simulink model "model_compatible"  (Simulink 7.5)
(part 3 of 3)

  金剛線_(Kongō_sen)_CN_109834508_275000_CN_291678103_275000 : powerlib/Elements/Distributed Parameters Line  Phases=3  Frequency=50  Resistance=[0.01273 0.3864]  Inductance="[0.9337e-3  4.1264e-3]"  Capacitance=[12.74e-9 7.751e-9]  Length=50.4928  x1=[8.73114913702011e-11 380000 380000;314.159265358979 314.159265358979 314.159265358979;-0.177670123217348 0.415246442777429 -1.15554988401747]  x2=[1.26090477118469e-09 381852.398472139 381852.398472139;314.159265358979 314.159265358979 314.159265358979;-1.41941675517191 0.415007521738739 -1.15578880505616]  x3=[1.07663708898761e-11 1405.24743813465 1405.24743813466;314.159265358979 314.159265358979 314.159265358979;-2.70558821102223 0.316110507002444 -1.25468581979246]  x4=[8.62234243168895e-12 1405.96374414071 1405.9637441407;314.159265358979 314.159265358979 314.159265358979;0.245769282942371 0.405640215255436 -1.16515611153945]  x5=0.000565541566995742  V1=ones(3,3)  V2=ones(3,3)  I1=ones(3,3)  I2=ones(3,3)  nHarmo=1  Measurements=None
  関門連系線_CN_204258596_500000_CN_187988970_500000 : powerlib/Elements/Distributed Parameters Line  Phases=3  Frequency=50  Resistance=[0.01273 0.3864]  Inductance="[0.9337e-3  4.1264e-3]"  Capacitance=[12.74e-9 7.751e-9]  Length=77.4957  x1=[8.73114913702011e-11 380000 380000;314.159265358979 314.159265358979 314.159265358979;-0.177670123217348 0.415246442777429 -1.15554988401747]  x2=[1.26090477118469e-09 381852.398472139 381852.398472139;314.159265358979 314.159265358979 314.159265358979;-1.41941675517191 0.415007521738739 -1.15578880505616]  x3=[1.07663708898761e-11 1405.24743813465 1405.24743813466;314.159265358979 314.159265358979 314.159265358979;-2.70558821102223 0.316110507002444 -1.25468581979246]  x4=[8.62234243168895e-12 1405.96374414071 1405.9637441407;314.159265358979 314.159265358979 314.159265358979;0.245769282942371 0.405640215255436 -1.16515611153945]  x5=0.000565541566995742  V1=ones(3,3)  V2=ones(3,3)  I1=ones(3,3)  I2=ones(3,3)  nHarmo=1  Measurements=None
  阿南紀北直流幹線_CN_109850439_500000_CN_217885658_500000 : powerlib/Elements/Distributed Parameters Line  Phases=3  Frequency=50  Resistance=[0.01273 0.3864]  Inductance="[0.9337e-3  4.1264e-3]"  Capacitance=[12.74e-9 7.751e-9]  Length=61.602  x1=[8.73114913702011e-11 380000 380000;314.159265358979 314.159265358979 314.159265358979;-0.177670123217348 0.415246442777429 -1.15554988401747]  x2=[1.26090477118469e-09 381852.398472139 381852.398472139;314.159265358979 314.159265358979 314.159265358979;-1.41941675517191 0.415007521738739 -1.15578880505616]  x3=[1.07663708898761e-11 1405.24743813465 1405.24743813466;314.159265358979 314.159265358979 314.159265358979;-2.70558821102223 0.316110507002444 -1.25468581979246]  x4=[8.62234243168895e-12 1405.96374414071 1405.9637441407;314.159265358979 314.159265358979 314.159265358979;0.245769282942371 0.405640215255436 -1.16515611153945]  x5=0.000565541566995742  V1=ones(3,3)  V2=ones(3,3)  I1=ones(3,3)  I2=ones(3,3)  nHarmo=1  Measurements=None
  駿遠幹線_CN_116559939_500000_CN_210090094_500000 : powerlib/Elements/Distributed Parameters Line  Phases=3  Frequency=50  Resistance=[0.01273 0.3864]  Inductance="[0.9337e-3  4.1264e-3]"  Capacitance=[12.74e-9 7.751e-9]  Length=56.5258  x1=[8.73114913702011e-11 380000 380000;314.159265358979 314.159265358979 314.159265358979;-0.177670123217348 0.415246442777429 -1.15554988401747]  x2=[1.26090477118469e-09 381852.398472139 381852.398472139;314.159265358979 314.159265358979 314.159265358979;-1.41941675517191 0.415007521738739 -1.15578880505616]  x3=[1.07663708898761e-11 1405.24743813465 1405.24743813466;314.159265358979 314.159265358979 314.159265358979;-2.70558821102223 0.316110507002444 -1.25468581979246]  x4=[8.62234243168895e-12 1405.96374414071 1405.9637441407;314.159265358979 314.159265358979 314.159265358979;0.245769282942371 0.405640215255436 -1.16515611153945]  x5=0.000565541566995742  V1=ones(3,3)  V2=ones(3,3)  I1=ones(3,3)  I2=ones(3,3)  nHarmo=1  Measurements=None
  connections:
  _CN_201293312_500000_CN_216778426_500000/LConn1 -- T_201293312_500000;220000_/LConn1 -- _CN_201293312_500000_CN_187988970_500000/LConn1
  _CN_201293312_500000_CN_216778426_500000/LConn2 -- T_201293312_500000;220000_/LConn2 -- _CN_201293312_500000_CN_187988970_500000/LConn2
  _CN_201293312_500000_CN_216778426_500000/LConn3 -- T_201293312_500000;220000_/LConn3 -- _CN_201293312_500000_CN_187988970_500000/LConn3
  T_216778426_500000;220000_/LConn1 -- _CN_201293312_500000_CN_216778426_500000/RConn1
  T_216778426_500000;220000_/LConn2 -- _CN_201293312_500000_CN_216778426_500000/RConn2
  T_216778426_500000;220000_/LConn3 -- _CN_201293312_500000_CN_216778426_500000/RConn3
  _CN_201293312_500000_CN_187988970_500000/RConn1 -- T_187988970_500000;220000_/LConn1 -- 関門連系線_CN_204258596_500000_CN_187988970_500000/LConn1
  _CN_201293312_500000_CN_187988970_500000/RConn2 -- T_187988970_500000;220000_/LConn2 -- 関門連系線_CN_204258596_500000_CN_187988970_500000/LConn2
  _CN_201293312_500000_CN_187988970_500000/RConn3 -- T_187988970_500000;220000_/LConn3 -- 関門連系線_CN_204258596_500000_CN_187988970_500000/LConn3
  T_169121281__北豊田変電所_(Kita_Toyota_Hendensho)/LConn1 -- _CN_169121281_275000_CN_169121284_275000/LConn1
  T_169121281__北豊田変電所_(Kita_Toyota_Hendensho)/LConn2 -- _CN_169121281_275000_CN_169121284_275000/LConn2
  T_169121281__北豊田変電所_(Kita_Toyota_Hendensho)/LConn3 -- _CN_169121281_275000_CN_169121284_275000/LConn3
  _CN_169121281_275000_CN_169121284_275000/RConn1 -- T_169121284_275000_/LConn1 -- _CN_169121284_275000_CN_169121278_275000/LConn1
  _CN_169121281_275000_CN_169121284_275000/RConn2 -- T_169121284_275000_/LConn2 -- _CN_169121284_275000_CN_169121278_275000/LConn2
  _CN_169121281_275000_CN_169121284_275000/RConn3 -- T_169121284_275000_/LConn3 -- _CN_169121284_275000_CN_169121278_275000/LConn3
  T_104173570_500000_/LConn1 -- _CN_104173570_500000_CN_106309481_500000/LConn1
  T_104173570_500000_/LConn2 -- _CN_104173570_500000_CN_106309481_500000/LConn2
  T_104173570_500000_/LConn3 -- _CN_104173570_500000_CN_106309481_500000/LConn3
  _CN_104173570_500000_CN_106309481_500000/RConn1 -- T_106309481_500000_新福島変電所/LConn1 -- 福島東幹線2_CN_106309481_500000_CN_104391636_500000/LConn1 -- _CN_106309481_500000_CN103783431/LConn1
  _CN_104173570_500000_CN_106309481_500000/RConn2 -- T_106309481_500000_新福島変電所/LConn2 -- 福島東幹線2_CN_106309481_500000_CN_104391636_500000/LConn2 -- _CN_106309481_500000_CN103783431/LConn2
  _CN_104173570_500000_CN_106309481_500000/RConn3 -- T_106309481_500000_新福島変電所/LConn3 -- 福島東幹線2_CN_106309481_500000_CN_104391636_500000/LConn3 -- _CN_106309481_500000_CN103783431/LConn3
  T_116828675_275000_北相模変電所_(Kita_Sagami_Hendensho)/LConn1 -- 佐久間東幹線_CN_116828675_275000_CN134376414/LConn1
  T_116828675_275000_北相模変電所_(Kita_Sagami_Hendensho)/LConn2 -- 佐久間東幹線_CN_116828675_275000_CN134376414/LConn2
  T_116828675_275000_北相模変電所_(Kita_Sagami_Hendensho)/LConn3 -- 佐久間東幹線_CN_116828675_275000_CN134376414/LConn3
  G_134376414_佐久間発電所/RConn1 -- 佐久間東幹線_CN_116828675_275000_CN134376414/RConn1
  G_134376414_佐久間発電所/RConn2 -- 佐久間東幹線_CN_116828675_275000_CN134376414/RConn2
  G_134376414_佐久間発電所/RConn3 -- 佐久間東幹線_CN_116828675_275000_CN134376414/RConn3
  _CN_169121284_275000_CN_169121278_275000/RConn1 -- T_169121278_275000_電源名古屋/LConn1 -- _CN_170366038_275000_CN_169121278_275000/LConn1
  _CN_169121284_275000_CN_169121278_275000/RConn2 -- T_169121278_275000_電源名古屋/LConn2 -- _CN_170366038_275000_CN_169121278_275000/LConn2
  _CN_169121284_275000_CN_169121278_275000/RConn3 -- T_169121278_275000_電源名古屋/LConn3 -- _CN_170366038_275000_CN_169121278_275000/LConn3
  T_170503689__/LConn1 -- _CN_170503689_275000_CN_170436908_275000/LConn1
  T_170503689__/LConn2 -- _CN_170503689_275000_CN_170436908_275000/LConn2
  T_170503689__/LConn3 -- _CN_170503689_275000_CN_170436908_275000/LConn3
  T_170436908__/LConn1 -- _CN_170503689_275000_CN_170436908_275000/RConn1
  T_170436908__/LConn2 -- _CN_170503689_275000_CN_170436908_275000/RConn2
  T_170436908__/LConn3 -- _CN_170503689_275000_CN_170436908_275000/RConn3
  T_168857610__/LConn1 -- _CN_168857610_500000_CN_104530060_500000/LConn1
  T_168857610__/LConn2 -- _CN_168857610_500000_CN_104530060_500000/LConn2
  T_168857610__/LConn3 -- _CN_168857610_500000_CN_104530060_500000/LConn3
  _CN_168857610_500000_CN_104530060_500000/RConn1 -- T_104530060__新栃木変電所/LConn1 -- _CN_104530060_500000_CN_315434358_500000/LConn1 -- _CN_104530060_500000_CN_168839127_500000/LConn1
  _CN_168857610_500000_CN_104530060_500000/RConn2 -- T_104530060__新栃木変電所/LConn2 -- _CN_104530060_500000_CN_315434358_500000/LConn2 -- _CN_104530060_500000_CN_168839127_500000/LConn2
  _CN_168857610_500000_CN_104530060_500000/RConn3 -- T_104530060__新栃木変電所/LConn3 -- _CN_104530060_500000_CN_315434358_500000/LConn3 -- _CN_104530060_500000_CN_168839127_500000/LConn3
  _CN_193544791_500000_CN_170974371_500000/LConn1 -- T_193544791_500000_新西広島変電所_(Shin_Nishi_Hiroshima_Hendensho)/LConn1 -- _CN_193544791_500000_CN_242253500_500000/LConn1 -- _CN_193544791_500000_CN_317416612_500000/LConn1
  _CN_193544791_500000_CN_170974371_500000/LConn2 -- T_193544791_500000_新西広島変電所_(Shin_Nishi_Hiroshima_Hendensho)/LConn2 -- _CN_193544791_500000_CN_242253500_500000/LConn2 -- _CN_193544791_500000_CN_317416612_500000/LConn2
  _CN_193544791_500000_CN_170974371_500000/LConn3 -- T_193544791_500000_新西広島変電所_(Shin_Nishi_Hiroshima_Hendensho)/LConn3 -- _CN_193544791_500000_CN_242253500_500000/LConn3 -- _CN_193544791_500000_CN_317416612_500000/LConn3
  _CN_193544791_500000_CN_170974371_500000/RConn1 -- T_170974371_500000_新広島変電所_(Shin_Hiroshima_Hendensho)/LConn1 -- _CN_170974371_500000_CN_241828221_500000/LConn1
  _CN_193544791_500000_CN_170974371_500000/RConn2 -- T_170974371_500000_新広島変電所_(Shin_Hiroshima_Hendensho)/LConn2 -- _CN_170974371_500000_CN_241828221_500000/LConn2
  _CN_193544791_500000_CN_170974371_500000/RConn3 -- T_170974371_500000_新広島変電所_(Shin_Hiroshima_Hendensho)/LConn3 -- _CN_170974371_500000_CN_241828221_500000/LConn3
  _CN_193544791_500000_CN_242253500_500000/RConn1 -- T_242253500_500000_東山口変電所_(Higashi_Yamaguchi_Hendensho)/LConn1 -- _CN_242253500_500000_CN_204258596_500000/LConn1
  _CN_193544791_500000_CN_242253500_500000/RConn2 -- T_242253500_500000_東山口変電所_(Higashi_Yamaguchi_Hendensho)/LConn2 -- _CN_242253500_500000_CN_204258596_500000/LConn2
  _CN_193544791_500000_CN_242253500_500000/RConn3 -- T_242253500_500000_東山口変電所_(Higashi_Yamaguchi_Hendensho)/LConn3 -- _CN_242253500_500000_CN_204258596_500000/LConn3
  _CN_193544791_500000_CN_317416612_500000/RConn1 -- T_317416612_500000_西島根変電所/LConn1 -- _CN_317416612_500000_CN_204258596_500000/LConn1 -- _CN_317416612_500000_CN_242103481_500000/LConn1
  _CN_193544791_500000_CN_317416612_500000/RConn2 -- T_317416612_500000_西島根変電所/LConn2 -- _CN_317416612_500000_CN_204258596_500000/LConn2 -- _CN_317416612_500000_CN_242103481_500000/LConn2
  _CN_193544791_500000_CN_317416612_500000/RConn3 -- T_317416612_500000_西島根変電所/LConn3 -- _CN_317416612_500000_CN_204258596_500000/LConn3 -- _CN_317416612_500000_CN_242103481_500000/LConn3
  _CN_161727149_500000_CN_169031921_500000/LConn1 -- T_161727149_500000_新生駒変電所_(Shin_Ikoma_Hendensho)/LConn1 -- _CN_161727149_500000_CN_161870227_500000/LConn1 -- _CN_161727149_500000_CN_169359724_500000/LConn1
  _CN_161727149_500000_CN_169031921_500000/LConn2 -- T_161727149_500000_新生駒変電所_(Shin_Ikoma_Hendensho)/LConn2 -- _CN_161727149_500000_CN_161870227_500000/LConn2 -- _CN_161727149_500000_CN_169359724_500000/LConn2
  _CN_161727149_500000_CN_169031921_500000/LConn3 -- T_161727149_500000_新生駒変電所_(Shin_Ikoma_Hendensho)/LConn3 -- _CN_161727149_500000_CN_161870227_500000/LConn3 -- _CN_161727149_500000_CN_169359724_500000/LConn3
  _CN_161727149_500000_CN_169031921_500000/RConn1 -- T_169031921_500000_西京都変電所_(Nishi_Kyōto_Hendensho)/LConn1 -- _CN_320438391_500000_CN_169031921_500000/LConn1
  _CN_161727149_500000_CN_169031921_500000/RConn2 -- T_169031921_500000_西京都変電所_(Nishi_Kyōto_Hendensho)/LConn2 -- _CN_320438391_500000_CN_169031921_500000/LConn2
  _CN_161727149_500000_CN_169031921_500000/RConn3 -- T_169031921_500000_西京都変電所_(Nishi_Kyōto_Hendensho)/LConn3 -- _CN_320438391_500000_CN_169031921_500000/LConn3
  T_169359724_500000_信貴変電所_(Shingi_Hendensho)/LConn1 -- _CN_161727149_500000_CN_169359724_500000/RConn1
  T_169359724_500000_信貴変電所_(Shingi_Hendensho)/LConn2 -- _CN_161727149_500000_CN_169359724_500000/RConn2
  T_169359724_500000_信貴変電所_(Shingi_Hendensho)/LConn3 -- _CN_161727149_500000_CN_169359724_500000/RConn3
  _CN_161727149_500000_CN_161870227_500000/RConn1 -- T_161870227_500000_南京都変電所_(Minami_Kyōto_Hendensho)/LConn1 -- _CN_170589736_500000_CN_161870227_500000/LConn1 -- _CN_169031998_500000_CN_161870227_500000/LConn1
  _CN_161727149_500000_CN_161870227_500000/RConn2 -- T_161870227_500000_南京都変電所_(Minami_Kyōto_Hendensho)/LConn2 -- _CN_170589736_500000_CN_161870227_500000/LConn2 -- _CN_169031998_500000_CN_161870227_500000/LConn2
  _CN_161727149_500000_CN_161870227_500000/RConn3 -- T_161870227_500000_南京都変電所_(Minami_Kyōto_Hendensho)/LConn3 -- _CN_170589736_500000_CN_161870227_500000/LConn3 -- _CN_169031998_500000_CN_161870227_500000/LConn3
  T_216502300__九州電力_中九州変電所/LConn1 -- 南九州幹線_CN_216502300_500000_CN_215451416_500000/LConn1
  T_216502300__九州電力_中九州変電所/LConn2 -- 南九州幹線_CN_216502300_500000_CN_215451416_500000/LConn2
  T_216502300__九州電力_中九州変電所/LConn3 -- 南九州幹線_CN_216502300_500000_CN_215451416_500000/LConn3
  南九州幹線_CN_216502300_500000_CN_215451416_500000/RConn1 -- T_215451416_500000;220000_九州電力南九州変電所/LConn1 -- _CN_215451416_500000_CN215429864/LConn1
  南九州幹線_CN_216502300_500000_CN_215451416_500000/RConn2 -- T_215451416_500000;220000_九州電力南九州変電所/LConn2 -- _CN_215451416_500000_CN215429864/LConn2
  南九州幹線_CN_216502300_500000_CN_215451416_500000/RConn3 -- T_215451416_500000;220000_九州電力南九州変電所/LConn3 -- _CN_215451416_500000_CN215429864/LConn3
  _CN_149843487_500000_CN_150065045_500000/LConn1 -- T_149843487_500000_新秦野変電所_(Shin_Hatano_Hendensho)/LConn1 -- 新多摩線_(Shin_Tama_Sen)_CN_149843487_500000_CN_145079972_500000/LConn1
  _CN_149843487_500000_CN_150065045_500000/LConn2 -- T_149843487_500000_新秦野変電所_(Shin_Hatano_Hendensho)/LConn2 -- 新多摩線_(Shin_Tama_Sen)_CN_149843487_500000_CN_145079972_500000/LConn2
  _CN_149843487_500000_CN_150065045_500000/LConn3 -- T_149843487_500000_新秦野変電所_(Shin_Hatano_Hendensho)/LConn3 -- 新多摩線_(Shin_Tama_Sen)_CN_149843487_500000_CN_145079972_500000/LConn3
  _CN_149843487_500000_CN_150065045_500000/RConn1 -- T_150065045_500000_新富士変電所/LConn1 -- _CN_150035494_500000_CN_150065045_500000/LConn1
  _CN_149843487_500000_CN_150065045_500000/RConn2 -- T_150065045_500000_新富士変電所/LConn2 -- _CN_150035494_500000_CN_150065045_500000/LConn2
  _CN_149843487_500000_CN_150065045_500000/RConn3 -- T_150065045_500000_新富士変電所/LConn3 -- _CN_150035494_500000_CN_150065045_500000/LConn3
  新多摩線_(Shin_Tama_Sen)_CN_149843487_500000_CN_145079972_500000/RConn1 -- T_145079972_500000_新多摩変電所_(Shin_Tama_Substation)/LConn1 -- 新所沢線_(Shin_Tokorozawa_Sen)_CN_133641619_500000_CN_145079972_500000/LConn1 -- _CN_195615141_500000_CN_145079972_500000/LConn1
  新多摩線_(Shin_Tama_Sen)_CN_149843487_500000_CN_145079972_500000/RConn2 -- T_145079972_500000_新多摩変電所_(Shin_Tama_Substation)/LConn2 -- 新所沢線_(Shin_Tokorozawa_Sen)_CN_133641619_500000_CN_145079972_500000/LConn2 -- _CN_195615141_500000_CN_145079972_500000/LConn2
  新多摩線_(Shin_Tama_Sen)_CN_149843487_500000_CN_145079972_500000/RConn3 -- T_145079972_500000_新多摩変電所_(Shin_Tama_Substation)/LConn3 -- 新所沢線_(Shin_Tokorozawa_Sen)_CN_133641619_500000_CN_145079972_500000/LConn3 -- _CN_195615141_500000_CN_145079972_500000/LConn3
  T_162844704_275000_中相模変電所/LConn1 -- 秦浜線_CN_162844704_275000_CN_128364781_275000/LConn1
  T_162844704_275000_中相模変電所/LConn2 -- 秦浜線_CN_162844704_275000_CN_128364781_275000/LConn2
  T_162844704_275000_中相模変電所/LConn3 -- 秦浜線_CN_162844704_275000_CN_128364781_275000/LConn3
  秦浜線_CN_162844704_275000_CN_128364781_275000/RConn1 -- T_128364781_275000_東京電力_京浜変電所/LConn1 -- 京浜線1;2号線_CN_128364781_275000_CN_47110637_275000/LConn1 -- 東京南線1;2号線_CN_128364781_275000_CN379474501/LConn1
  秦浜線_CN_162844704_275000_CN_128364781_275000/RConn2 -- T_128364781_275000_東京電力_京浜変電所/LConn2 -- 京浜線1;2号線_CN_128364781_275000_CN_47110637_275000/LConn2 -- 東京南線1;2号線_CN_128364781_275000_CN379474501/LConn2
  秦浜線_CN_162844704_275000_CN_128364781_275000/RConn3 -- T_128364781_275000_東京電力_京浜変電所/LConn3 -- 京浜線1;2号線_CN_128364781_275000_CN_47110637_275000/LConn3 -- 東京南線1;2号線_CN_128364781_275000_CN379474501/LConn3
  _CN_150035494_500000_CN216480979/LConn1 -- T_150035494_500000_/LConn1 -- _CN_150035494_500000_CN_341208725_500000/LConn1 -- _CN_150035494_500000_CN_150065045_500000/RConn1 -- _CN_150035494_500000_CN_66098469_500000/LConn1
  _CN_150035494_500000_CN216480979/LConn2 -- T_150035494_500000_/LConn2 -- _CN_150035494_500000_CN_341208725_500000/LConn2 -- _CN_150035494_500000_CN_150065045_500000/RConn2 -- _CN_150035494_500000_CN_66098469_500000/LConn2
  _CN_150035494_500000_CN216480979/LConn3 -- T_150035494_500000_/LConn3 -- _CN_150035494_500000_CN_341208725_500000/LConn3 -- _CN_150035494_500000_CN_150065045_500000/RConn3 -- _CN_150035494_500000_CN_66098469_500000/LConn3
  _CN_150035494_500000_CN216480979/RConn1 -- G_216480979_柏崎刈羽原子力発電所/RConn1 -- _CN_66098469_500000_CN216480979/LConn1
  _CN_150035494_500000_CN216480979/RConn2 -- G_216480979_柏崎刈羽原子力発電所/RConn2 -- _CN_66098469_500000_CN216480979/LConn2
  _CN_150035494_500000_CN216480979/RConn3 -- G_216480979_柏崎刈羽原子力発電所/RConn3 -- _CN_66098469_500000_CN216480979/LConn3
  _CN_150035494_500000_CN_66098469_500000/RConn1 -- T_66098469_500000_西群馬開閉所/LConn1 -- 東群馬幹線_CN_250540807_500000_CN_66098469_500000/LConn1 -- _CN_66098469_500000_CN216480979/RConn1 -- 新吾妻線_CN_169963236_500000_CN_66098469_500000/LConn1
  _CN_150035494_500000_CN_66098469_500000/RConn2 -- T_66098469_500000_西群馬開閉所/LConn2 -- 東群馬幹線_CN_250540807_500000_CN_66098469_500000/LConn2 -- _CN_66098469_500000_CN216480979/RConn2 -- 新吾妻線_CN_169963236_500000_CN_66098469_500000/LConn2
  _CN_150035494_500000_CN_66098469_500000/RConn3 -- T_66098469_500000_西群馬開閉所/LConn3 -- 東群馬幹線_CN_250540807_500000_CN_66098469_500000/LConn3 -- _CN_66098469_500000_CN216480979/RConn3 -- 新吾妻線_CN_169963236_500000_CN_66098469_500000/LConn3
  T_341208725__/LConn1 -- _CN_150035494_500000_CN_341208725_500000/RConn1
  T_341208725__/LConn2 -- _CN_150035494_500000_CN_341208725_500000/RConn2
  T_341208725__/LConn3 -- _CN_150035494_500000_CN_341208725_500000/RConn3
  _CN_340647463_275000_CN_340648895_275000/LConn1 -- T_340647463__/LConn1 -- _CN_340647463_275000_CN_168852840_275000/LConn1 -- _CN_340647463_275000_CN_340647468_275000/LConn1
  _CN_340647463_275000_CN_340648895_275000/LConn2 -- T_340647463__/LConn2 -- _CN_340647463_275000_CN_168852840_275000/LConn2 -- _CN_340647463_275000_CN_340647468_275000/LConn2
  _CN_340647463_275000_CN_340648895_275000/LConn3 -- T_340647463__/LConn3 -- _CN_340647463_275000_CN_168852840_275000/LConn3 -- _CN_340647463_275000_CN_340647468_275000/LConn3
  T_340648895__/LConn1 -- _CN_340647463_275000_CN_340648895_275000/RConn1
  T_340648895__/LConn2 -- _CN_340647463_275000_CN_340648895_275000/RConn2
  T_340648895__/LConn3 -- _CN_340647463_275000_CN_340648895_275000/RConn3
  _CN_340647463_275000_CN_168852840_275000/RConn1 -- T_168852840__/LConn1 -- 新京葉線_CN_151706977_275000_CN_168852840_275000/LConn1
  _CN_340647463_275000_CN_168852840_275000/RConn2 -- T_168852840__/LConn2 -- 新京葉線_CN_151706977_275000_CN_168852840_275000/LConn2
  _CN_340647463_275000_CN_168852840_275000/RConn3 -- T_168852840__/LConn3 -- 新京葉線_CN_151706977_275000_CN_168852840_275000/LConn3
  T_340647468__/LConn1 -- _CN_340647463_275000_CN_340647468_275000/RConn1
  T_340647468__/LConn2 -- _CN_340647463_275000_CN_340647468_275000/RConn2
  T_340647468__/LConn3 -- _CN_340647463_275000_CN_340647468_275000/RConn3
  _CN_170589736_500000_CN_161870227_500000/RConn1 -- T_170589736_500000_東近江/LConn1 -- _CN_170589736_500000_CN_170568495_500000/LConn1
  _CN_170589736_500000_CN_161870227_500000/RConn2 -- T_170589736_500000_東近江/LConn2 -- _CN_170589736_500000_CN_170568495_500000/LConn2
  _CN_170589736_500000_CN_161870227_500000/RConn3 -- T_170589736_500000_東近江/LConn3 -- _CN_170589736_500000_CN_170568495_500000/LConn3
  _CN_170589736_500000_CN_170568495_500000/RConn1 -- T_170568495_500000_三重開閉所/LConn1 -- _CN_170537514_500000_CN_170568495_500000/LConn1 -- _CN_170366035_500000_CN_170568495_500000/LConn1
  _CN_170589736_500000_CN_170568495_500000/RConn2 -- T_170568495_500000_三重開閉所/LConn2 -- _CN_170537514_500000_CN_170568495_500000/LConn2 -- _CN_170366035_500000_CN_170568495_500000/LConn2
  _CN_170589736_500000_CN_170568495_500000/RConn3 -- T_170568495_500000_三重開閉所/LConn3 -- _CN_170537514_500000_CN_170568495_500000/LConn3 -- _CN_170366035_500000_CN_170568495_500000/LConn3
  T_319300956_275000_中越変電所/LConn1 -- _CN_319300956_275000_CN_318218831_275000/LConn1
  T_319300956_275000_中越変電所/LConn2 -- _CN_319300956_275000_CN_318218831_275000/LConn2
  T_319300956_275000_中越変電所/LConn3 -- _CN_319300956_275000_CN_318218831_275000/LConn3
  _CN_319300956_275000_CN_318218831_275000/RConn1 -- T_318218831_275000_/LConn1 -- _CN_318218831_275000_CN_169993955_275000/LConn1 -- _CN_318218831_275000_CN_170016148_275000/LConn1 -- _CN_103818820_275000_CN_318218831_275000/LConn1
  _CN_319300956_275000_CN_318218831_275000/RConn2 -- T_318218831_275000_/LConn2 -- _CN_318218831_275000_CN_169993955_275000/LConn2 -- _CN_318218831_275000_CN_170016148_275000/LConn2 -- _CN_103818820_275000_CN_318218831_275000/LConn2
  _CN_319300956_275000_CN_318218831_275000/RConn3 -- T_318218831_275000_/LConn3 -- _CN_318218831_275000_CN_169993955_275000/LConn3 -- _CN_318218831_275000_CN_170016148_275000/LConn3 -- _CN_103818820_275000_CN_318218831_275000/LConn3
  _CN_170537514_500000_CN_161946849_500000/LConn1 -- T_170537514_500000_/LConn1 -- _CN_170537514_500000_CN_170568495_500000/RConn1
  _CN_170537514_500000_CN_161946849_500000/LConn2 -- T_170537514_500000_/LConn2 -- _CN_170537514_500000_CN_170568495_500000/RConn2
  _CN_170537514_500000_CN_161946849_500000/LConn3 -- T_170537514_500000_/LConn3 -- _CN_170537514_500000_CN_170568495_500000/RConn3
  _CN_170537514_500000_CN_161946849_500000/RConn1 -- T_161946849_500000;275000_北部変電所/LConn1 -- _CN_169122898_500000_CN_161946849_500000/LConn1 -- _CN_170366035_500000_CN_161946849_500000/LConn1
  _CN_170537514_500000_CN_161946849_500000/RConn2 -- T_161946849_500000;275000_北部変電所/LConn2 -- _CN_169122898_500000_CN_161946849_500000/LConn2 -- _CN_170366035_500000_CN_161946849_500000/LConn2
  _CN_170537514_500000_CN_161946849_500000/RConn3 -- T_161946849_500000;275000_北部変電所/LConn3 -- _CN_169122898_500000_CN_161946849_500000/LConn3 -- _CN_170366035_500000_CN_161946849_500000/LConn3
  T_192745005_275000_丸山変電所_(Maruyama_Hendensho)/LConn1 -- 丸山幹線_(Maruyama_Kansen)_CN_192745005_275000_CN_161946848_275000/LConn1
  T_192745005_275000_丸山変電所_(Maruyama_Hendensho)/LConn2 -- 丸山幹線_(Maruyama_Kansen)_CN_192745005_275000_CN_161946848_275000/LConn2
  T_192745005_275000_丸山変電所_(Maruyama_Hendensho)/LConn3 -- 丸山幹線_(Maruyama_Kansen)_CN_192745005_275000_CN_161946848_275000/LConn3
  丸山幹線_(Maruyama_Kansen)_CN_192745005_275000_CN_161946848_275000/RConn1 -- T_161946848_275000_関開閉所_(Seki)/LConn1 -- _CN_161946848_275000_CN_190734269_275000/LConn1
  丸山幹線_(Maruyama_Kansen)_CN_192745005_275000_CN_161946848_275000/RConn2 -- T_161946848_275000_関開閉所_(Seki)/LConn2 -- _CN_161946848_275000_CN_190734269_275000/LConn2
  丸山幹線_(Maruyama_Kansen)_CN_192745005_275000_CN_161946848_275000/RConn3 -- T_161946848_275000_関開閉所_(Seki)/LConn3 -- _CN_161946848_275000_CN_190734269_275000/LConn3
  _CN_108199478_275000_CN_109834508_275000/LConn1 -- T_108199478_275000_南大阪変電所_(Minamiōsaka_Hendensho)/LConn1 -- 泉南東大阪線_(Sennan_Higashiōsaka_sen)_CN_108199478_275000_CN_158522649_275000/LConn1
  _CN_108199478_275000_CN_109834508_275000/LConn2 -- T_108199478_275000_南大阪変電所_(Minamiōsaka_Hendensho)/LConn2 -- 泉南東大阪線_(Sennan_Higashiōsaka_sen)_CN_108199478_275000_CN_158522649_275000/LConn2
  _CN_108199478_275000_CN_109834508_275000/LConn3 -- T_108199478_275000_南大阪変電所_(Minamiōsaka_Hendensho)/LConn3 -- 泉南東大阪線_(Sennan_Higashiōsaka_sen)_CN_108199478_275000_CN_158522649_275000/LConn3
  _CN_108199478_275000_CN_109834508_275000/RConn1 -- T_109834508_275000_金剛開閉所_(Kongō_Kaiheisho)/LConn1 -- 北葛城線_(Kita_Katsuragi_Sen)_CN_160374974_275000_CN_109834508_275000/LConn1 -- 金剛線_(Kongō_sen)_CN_109834508_275000_CN_291678103_275000/LConn1
  _CN_108199478_275000_CN_109834508_275000/RConn2 -- T_109834508_275000_金剛開閉所_(Kongō_Kaiheisho)/LConn2 -- 北葛城線_(Kita_Katsuragi_Sen)_CN_160374974_275000_CN_109834508_275000/LConn2 -- 金剛線_(Kongō_sen)_CN_109834508_275000_CN_291678103_275000/LConn2
  _CN_108199478_275000_CN_109834508_275000/RConn3 -- T_109834508_275000_金剛開閉所_(Kongō_Kaiheisho)/LConn3 -- 北葛城線_(Kita_Katsuragi_Sen)_CN_160374974_275000_CN_109834508_275000/LConn3 -- 金剛線_(Kongō_sen)_CN_109834508_275000_CN_291678103_275000/LConn3
  T_158522649_275000_東大阪変電所/LConn1 -- 泉南東大阪線_(Sennan_Higashiōsaka_sen)_CN_108199478_275000_CN_158522649_275000/RConn1
  T_158522649_275000_東大阪変電所/LConn2 -- 泉南東大阪線_(Sennan_Higashiōsaka_sen)_CN_108199478_275000_CN_158522649_275000/RConn2
  T_158522649_275000_東大阪変電所/LConn3 -- 泉南東大阪線_(Sennan_Higashiōsaka_sen)_CN_108199478_275000_CN_158522649_275000/RConn3
  T_315614776_275000_/LConn1 -- _CN_315614776_275000_CN_315614783_275000/LConn1
  T_315614776_275000_/LConn2 -- _CN_315614776_275000_CN_315614783_275000/LConn2
  T_315614776_275000_/LConn3 -- _CN_315614776_275000_CN_315614783_275000/LConn3
  _CN_315614776_275000_CN_315614783_275000/RConn1 -- T_315614783_275000_/LConn1 -- _CN_315614783_275000_CN_256682313_275000/LConn1
  _CN_315614776_275000_CN_315614783_275000/RConn2 -- T_315614783_275000_/LConn2 -- _CN_315614783_275000_CN_256682313_275000/LConn2
  _CN_315614776_275000_CN_315614783_275000/RConn3 -- T_315614783_275000_/LConn3 -- _CN_315614783_275000_CN_256682313_275000/LConn3
  T_316566585_275000_/LConn1 -- _CN_316566585_275000_CN_174636874_275000/LConn1
  T_316566585_275000_/LConn2 -- _CN_316566585_275000_CN_174636874_275000/LConn2
  T_316566585_275000_/LConn3 -- _CN_316566585_275000_CN_174636874_275000/LConn3
  _CN_316566585_275000_CN_174636874_275000/RConn1 -- T_174636874_275000_岩手変電所/LConn1 -- _CN_316566588_275000_CN_174636874_275000/LConn1
  _CN_316566585_275000_CN_174636874_275000/RConn2 -- T_174636874_275000_岩手変電所/LConn2 -- _CN_316566588_275000_CN_174636874_275000/LConn2
  _CN_316566585_275000_CN_174636874_275000/RConn3 -- T_174636874_275000_岩手変電所/LConn3 -- _CN_316566588_275000_CN_174636874_275000/LConn3
  _CN_316566588_275000_CN_316581632_275000/LConn1 -- T_316566588_275000_/LConn1 -- _CN_316566588_275000_CN_308348224_275000/LConn1 -- _CN_316566588_275000_CN_174636874_275000/RConn1
  _CN_316566588_275000_CN_316581632_275000/LConn2 -- T_316566588_275000_/LConn2 -- _CN_316566588_275000_CN_308348224_275000/LConn2 -- _CN_316566588_275000_CN_174636874_275000/RConn2
  _CN_316566588_275000_CN_316581632_275000/LConn3 -- T_316566588_275000_/LConn3 -- _CN_316566588_275000_CN_308348224_275000/LConn3 -- _CN_316566588_275000_CN_174636874_275000/RConn3
  T_316581632_275000_/LConn1 -- _CN_316566588_275000_CN_316581632_275000/RConn1
  T_316581632_275000_/LConn2 -- _CN_316566588_275000_CN_316581632_275000/RConn2
  T_316581632_275000_/LConn3 -- _CN_316566588_275000_CN_316581632_275000/RConn3
  T_308348224_275000_新庄変電所/LConn1 -- _CN_316566588_275000_CN_308348224_275000/RConn1
  T_308348224_275000_新庄変電所/LConn2 -- _CN_316566588_275000_CN_308348224_275000/RConn2
  T_308348224_275000_新庄変電所/LConn3 -- _CN_316566588_275000_CN_308348224_275000/RConn3
  _CN_315614783_275000_CN_256682313_275000/RConn1 -- T_256682313__/LConn1 -- _CN_315757225_275000_CN_256682313_275000/LConn1
  _CN_315614783_275000_CN_256682313_275000/RConn2 -- T_256682313__/LConn2 -- _CN_315757225_275000_CN_256682313_275000/LConn2
  _CN_315614783_275000_CN_256682313_275000/RConn3 -- T_256682313__/LConn3 -- _CN_315757225_275000_CN_256682313_275000/LConn3
  T_116559939_500000_/LConn1 -- 駿遠幹線_CN_116559939_500000_CN_210090094_500000/LConn1
  T_116559939_500000_/LConn2 -- 駿遠幹線_CN_116559939_500000_CN_210090094_500000/LConn2
  T_116559939_500000_/LConn3 -- 駿遠幹線_CN_116559939_500000_CN_210090094_500000/LConn3
  T_210090094_500000_駿遠変電所/LConn1 -- 駿遠幹線_CN_116559939_500000_CN_210090094_500000/RConn1
  T_210090094_500000_駿遠変電所/LConn2 -- 駿遠幹線_CN_116559939_500000_CN_210090094_500000/RConn2
  T_210090094_500000_駿遠変電所/LConn3 -- 駿遠幹線_CN_116559939_500000_CN_210090094_500000/RConn3
  _CN_103818820_275000_CN_318218831_275000/RConn1 -- T_103818820_275000_仙台変電所/LConn1 -- _CN_103818820_275000_CN_250430935_275000/LConn1
  _CN_103818820_275000_CN_318218831_275000/RConn2 -- T_103818820_275000_仙台変電所/LConn2 -- _CN_103818820_275000_CN_250430935_275000/LConn2
  _CN_103818820_275000_CN_318218831_275000/RConn3 -- T_103818820_275000_仙台変電所/LConn3 -- _CN_103818820_275000_CN_250430935_275000/LConn3
  _CN_103818820_275000_CN_250430935_275000/RConn1 -- T_250430935_275000_米沢変電所_(Yonezawa_Hendensho)/LConn1 -- _CN_250430935_275000_CN_107262429_275000/LConn1 -- _CN_169993955_275000_CN_250430935_275000/LConn1 -- _CN_250430935_275000_CN354115662/LConn1
  _CN_103818820_275000_CN_250430935_275000/RConn2 -- T_250430935_275000_米沢変電所_(Yonezawa_Hendensho)/LConn2 -- _CN_250430935_275000_CN_107262429_275000/LConn2 -- _CN_169993955_275000_CN_250430935_275000/LConn2 -- _CN_250430935_275000_CN354115662/LConn2
  _CN_103818820_275000_CN_250430935_275000/RConn3 -- T_250430935_275000_米沢変電所_(Yonezawa_Hendensho)/LConn3 -- _CN_250430935_275000_CN_107262429_275000/LConn3 -- _CN_169993955_275000_CN_250430935_275000/LConn3 -- _CN_250430935_275000_CN354115662/LConn3
  T_172601929_500000;220000_/LConn1 -- _CN_172601929_500000_CN_186510275_500000/LConn1
  T_172601929_500000;220000_/LConn2 -- _CN_172601929_500000_CN_186510275_500000/LConn2
  T_172601929_500000;220000_/LConn3 -- _CN_172601929_500000_CN_186510275_500000/LConn3
  T_186510275_500000_3_4号_開閉所/LConn1 -- _CN_172601929_500000_CN_186510275_500000/RConn1
  T_186510275_500000_3_4号_開閉所/LConn2 -- _CN_172601929_500000_CN_186510275_500000/RConn2
  T_186510275_500000_3_4号_開閉所/LConn3 -- _CN_172601929_500000_CN_186510275_500000/RConn3
  T_327974991__東京電力逗子変電所/LConn1 -- 逗子線_CN_327974991_275000_CN379474501/LConn1
  T_327974991__東京電力逗子変電所/LConn2 -- 逗子線_CN_327974991_275000_CN379474501/LConn2
  T_327974991__東京電力逗子変電所/LConn3 -- 逗子線_CN_327974991_275000_CN379474501/LConn3
  逗子線_CN_327974991_275000_CN379474501/RConn1 -- G_379474501_/RConn1 -- 東京南線1;2号線_CN_128364781_275000_CN379474501/RConn1
  逗子線_CN_327974991_275000_CN379474501/RConn2 -- G_379474501_/RConn2 -- 東京南線1;2号線_CN_128364781_275000_CN379474501/RConn2
  逗子線_CN_327974991_275000_CN379474501/RConn3 -- G_379474501_/RConn3 -- 東京南線1;2号線_CN_128364781_275000_CN379474501/RConn3
  _CN_158064651_275000_CN_232998815_275000/LConn1 -- T_158064651_275000_田子倉発電所/LConn1 -- _CN_158064651_275000_CN319098734/LConn1
  _CN_158064651_275000_CN_232998815_275000/LConn2 -- T_158064651_275000_田子倉発電所/LConn2 -- _CN_158064651_275000_CN319098734/LConn2
  _CN_158064651_275000_CN_232998815_275000/LConn3 -- T_158064651_275000_田子倉発電所/LConn3 -- _CN_158064651_275000_CN319098734/LConn3
  _CN_158064651_275000_CN_232998815_275000/RConn1 -- T_232998815_275000_/LConn1 -- _CN_232998815_275000_CN233174201/LConn1
  _CN_158064651_275000_CN_232998815_275000/RConn2 -- T_232998815_275000_/LConn2 -- _CN_232998815_275000_CN233174201/LConn2
  _CN_158064651_275000_CN_232998815_275000/RConn3 -- T_232998815_275000_/LConn3 -- _CN_232998815_275000_CN233174201/LConn3
  _CN_158064651_275000_CN319098734/RConn1 -- G_319098734_信濃川水力発電所/RConn1 -- _CN_318302348_275000_CN319098734/LConn1
  _CN_158064651_275000_CN319098734/RConn2 -- G_319098734_信濃川水力発電所/RConn2 -- _CN_318302348_275000_CN319098734/LConn2
  _CN_158064651_275000_CN319098734/RConn3 -- G_319098734_信濃川水力発電所/RConn3 -- _CN_318302348_275000_CN319098734/LConn3
  _CN_169122898_500000_CN_161946849_500000/RConn1 -- T_169122898_500000_東部変電所/LConn1 -- _CN_169122898_500000_CN_142662111_500000/LConn1 -- _CN_169122898_500000_CN_170247312_500000/LConn1
  _CN_169122898_500000_CN_161946849_500000/RConn2 -- T_169122898_500000_東部変電所/LConn2 -- _CN_169122898_500000_CN_142662111_500000/LConn2 -- _CN_169122898_500000_CN_170247312_500000/LConn2
  _CN_169122898_500000_CN_161946849_500000/RConn3 -- T_169122898_500000_東部変電所/LConn3 -- _CN_169122898_500000_CN_142662111_500000/LConn3 -- _CN_169122898_500000_CN_170247312_500000/LConn3
  T_170247312_500000_新三河/LConn1 -- _CN_169122898_500000_CN_170247312_500000/RConn1
  T_170247312_500000_新三河/LConn2 -- _CN_169122898_500000_CN_170247312_500000/RConn2
  T_170247312_500000_新三河/LConn3 -- _CN_169122898_500000_CN_170247312_500000/RConn3
  _CN_169122898_500000_CN_142662111_500000/RConn1 -- T_142662111_500000_中部電力㈱豊根開閉所/LConn1 -- 南信幹線_CN_209429410_500000_CN_142662111_500000/LConn1 -- 豊根幹線_CN_142662111_500000_CN_170850727_500000/LConn1
  _CN_169122898_500000_CN_142662111_500000/RConn2 -- T_142662111_500000_中部電力㈱豊根開閉所/LConn2 -- 南信幹線_CN_209429410_500000_CN_142662111_500000/LConn2 -- 豊根幹線_CN_142662111_500000_CN_170850727_500000/LConn2
  _CN_169122898_500000_CN_142662111_500000/RConn3 -- T_142662111_500000_中部電力㈱豊根開閉所/LConn3 -- 南信幹線_CN_209429410_500000_CN_142662111_500000/LConn3 -- 豊根幹線_CN_142662111_500000_CN_170850727_500000/LConn3
  _CN_170366035_500000_CN_170568495_500000/RConn1 -- T_170366035_500000_/LConn1 -- _CN_170366035_500000_CN_170850727_500000/LConn1 -- _CN_170366035_500000_CN_161946849_500000/RConn1
  _CN_170366035_500000_CN_170568495_500000/RConn2 -- T_170366035_500000_/LConn2 -- _CN_170366035_500000_CN_170850727_500000/LConn2 -- _CN_170366035_500000_CN_161946849_500000/RConn2
  _CN_170366035_500000_CN_170568495_500000/RConn3 -- T_170366035_500000_/LConn3 -- _CN_170366035_500000_CN_170850727_500000/LConn3 -- _CN_170366035_500000_CN_161946849_500000/RConn3
  _CN_170366035_500000_CN_170850727_500000/RConn1 -- T_170850727_500000_愛知変電所/LConn1 -- 豊根幹線_CN_142662111_500000_CN_170850727_500000/RConn1
  _CN_170366035_500000_CN_170850727_500000/RConn2 -- T_170850727_500000_愛知変電所/LConn2 -- 豊根幹線_CN_142662111_500000_CN_170850727_500000/RConn2
  _CN_170366035_500000_CN_170850727_500000/RConn3 -- T_170850727_500000_愛知変電所/LConn3 -- 豊根幹線_CN_142662111_500000_CN_170850727_500000/RConn3
  T_170366036_275000_東豊田変電所/LConn1 -- _CN_170366036_275000_CN_170247359_275000/LConn1
  T_170366036_275000_東豊田変電所/LConn2 -- _CN_170366036_275000_CN_170247359_275000/LConn2
  T_170366036_275000_東豊田変電所/LConn3 -- _CN_170366036_275000_CN_170247359_275000/LConn3
  _CN_170366036_275000_CN_170247359_275000/RConn1 -- T_170247359_275000_/LConn1 -- _CN_170247314_275000_CN_170247359_275000/LConn1
  _CN_170366036_275000_CN_170247359_275000/RConn2 -- T_170247359_275000_/LConn2 -- _CN_170247314_275000_CN_170247359_275000/LConn2
  _CN_170366036_275000_CN_170247359_275000/RConn3 -- T_170247359_275000_/LConn3 -- _CN_170247314_275000_CN_170247359_275000/LConn3
  _CN_170366038_275000_CN_161946849_275000/LConn1 -- T_170366038_275000_/LConn1 -- _CN_170366038_275000_CN_169121278_275000/RConn1
  _CN_170366038_275000_CN_161946849_275000/LConn2 -- T_170366038_275000_/LConn2 -- _CN_170366038_275000_CN_169121278_275000/RConn2
  _CN_170366038_275000_CN_161946849_275000/LConn3 -- T_170366038_275000_/LConn3 -- _CN_170366038_275000_CN_169121278_275000/RConn3
  _CN_170366038_275000_CN_161946849_275000/RConn1 -- T_161946849_500000;275000_北部変電所/RConn1 -- _CN_161946849_275000_CN_161948515_275000/LConn1 -- _CN_161946849_275000_CN210658603/LConn1 -- L_161946849/LConn1
  _CN_170366038_275000_CN_161946849_275000/RConn2 -- T_161946849_500000;275000_北部変電所/RConn2 -- _CN_161946849_275000_CN_161948515_275000/LConn2 -- _CN_161946849_275000_CN210658603/LConn2 -- L_161946849/LConn2
  _CN_170366038_275000_CN_161946849_275000/RConn3 -- T_161946849_500000;275000_北部変電所/RConn3 -- _CN_161946849_275000_CN_161948515_275000/LConn3 -- _CN_161946849_275000_CN210658603/LConn3 -- L_161946849/LConn3
  _CN_241956440_275000_CN214992492/LConn1 -- T_241956440_275000_伊勢開閉所/LConn1 -- _CN_241956440_275000_CN_241923317_275000/LConn1 -- _CN_241956440_275000_CN_242532736_275000/LConn1 -- 伊勢幹線_CN_241956440_275000_CN_170793703_275000/LConn1
  _CN_241956440_275000_CN214992492/LConn2 -- T_241956440_275000_伊勢開閉所/LConn2 -- _CN_241956440_275000_CN_241923317_275000/LConn2 -- _CN_241956440_275000_CN_242532736_275000/LConn2 -- 伊勢幹線_CN_241956440_275000_CN_170793703_275000/LConn2
  _CN_241956440_275000_CN214992492/LConn3 -- T_241956440_275000_伊勢開閉所/LConn3 -- _CN_241956440_275000_CN_241923317_275000/LConn3 -- _CN_241956440_275000_CN_242532736_275000/LConn3 -- 伊勢幹線_CN_241956440_275000_CN_170793703_275000/LConn3
  G_214992492_/RConn1 -- _CN_241956440_275000_CN214992492/RConn1
  G_214992492_/RConn2 -- _CN_241956440_275000_CN214992492/RConn2
  G_214992492_/RConn3 -- _CN_241956440_275000_CN214992492/RConn3
  T_242532736_275000_/LConn1 -- _CN_241956440_275000_CN_242532736_275000/RConn1
  T_242532736_275000_/LConn2 -- _CN_241956440_275000_CN_242532736_275000/RConn2
  T_242532736_275000_/LConn3 -- _CN_241956440_275000_CN_242532736_275000/RConn3
  伊勢幹線_CN_241956440_275000_CN_170793703_275000/RConn1 -- T_170793703_275000_西尾張/LConn1 -- _CN_170793702_275000_CN_170793703_275000/LConn1 -- _CN_262597734_275000_CN_170793703_275000/LConn1
  伊勢幹線_CN_241956440_275000_CN_170793703_275000/RConn2 -- T_170793703_275000_西尾張/LConn2 -- _CN_170793702_275000_CN_170793703_275000/LConn2 -- _CN_262597734_275000_CN_170793703_275000/LConn2
  伊勢幹線_CN_241956440_275000_CN_170793703_275000/RConn3 -- T_170793703_275000_西尾張/LConn3 -- _CN_170793702_275000_CN_170793703_275000/LConn3 -- _CN_262597734_275000_CN_170793703_275000/LConn3
  T_241923317_275000_南勢変電所_(Nansei_Hendensho)/LConn1 -- _CN_241956440_275000_CN_241923317_275000/RConn1
  T_241923317_275000_南勢変電所_(Nansei_Hendensho)/LConn2 -- _CN_241956440_275000_CN_241923317_275000/RConn2
  T_241923317_275000_南勢変電所_(Nansei_Hendensho)/LConn3 -- _CN_241956440_275000_CN_241923317_275000/RConn3
  _CN_318218831_275000_CN_169993955_275000/RConn1 -- T_169993955_275000_新潟変電所/LConn1 -- _CN_169993955_275000_CN_250430935_275000/RConn1
  _CN_318218831_275000_CN_169993955_275000/RConn2 -- T_169993955_275000_新潟変電所/LConn2 -- _CN_169993955_275000_CN_250430935_275000/RConn2
  _CN_318218831_275000_CN_169993955_275000/RConn3 -- T_169993955_275000_新潟変電所/LConn3 -- _CN_169993955_275000_CN_250430935_275000/RConn3
  T_170016148_275000_北新潟変電所/LConn1 -- _CN_318218831_275000_CN_170016148_275000/RConn1
  T_170016148_275000_北新潟変電所/LConn2 -- _CN_318218831_275000_CN_170016148_275000/RConn2
  T_170016148_275000_北新潟変電所/LConn3 -- _CN_318218831_275000_CN_170016148_275000/RConn3
  東京中線_CN_133137636_275000_CN_128581912_275000/LConn1 -- T_133137636_275000_北東京変電所_(Kita_Tōkyō_Hendensho)/LConn1 -- 東京北線_(Tōkyō_Kita_Sen)_CN_133137636_275000_CN_151706977_275000/LConn1 -- 西越谷線_(Nishi_Koshigaya_Sen)_CN_133137636_275000_CN_155411568_275000/LConn1
  東京中線_CN_133137636_275000_CN_128581912_275000/LConn2 -- T_133137636_275000_北東京変電所_(Kita_Tōkyō_Hendensho)/LConn2 -- 東京北線_(Tōkyō_Kita_Sen)_CN_133137636_275000_CN_151706977_275000/LConn2 -- 西越谷線_(Nishi_Koshigaya_Sen)_CN_133137636_275000_CN_155411568_275000/LConn2
  東京中線_CN_133137636_275000_CN_128581912_275000/LConn3 -- T_133137636_275000_北東京変電所_(Kita_Tōkyō_Hendensho)/LConn3 -- 東京北線_(Tōkyō_Kita_Sen)_CN_133137636_275000_CN_151706977_275000/LConn3 -- 西越谷線_(Nishi_Koshigaya_Sen)_CN_133137636_275000_CN_155411568_275000/LConn3
  東京中線_CN_133137636_275000_CN_128581912_275000/RConn1 -- T_128581912_500000;275000;66000_新坂戸変電所/RConn1 -- _CN_87682157_275000_CN_128581912_275000/LConn1
  東京中線_CN_133137636_275000_CN_128581912_275000/RConn2 -- T_128581912_500000;275000;66000_新坂戸変電所/RConn2 -- _CN_87682157_275000_CN_128581912_275000/LConn2
  東京中線_CN_133137636_275000_CN_128581912_275000/RConn3 -- T_128581912_500000;275000;66000_新坂戸変電所/RConn3 -- _CN_87682157_275000_CN_128581912_275000/LConn3
  東京北線_(Tōkyō_Kita_Sen)_CN_133137636_275000_CN_151706977_275000/RConn1 -- T_151706977__新野田変電所_(Shin_Noda_Hendensho)/RConn1 -- 新京葉線_CN_151706977_275000_CN_168852840_275000/RConn1 -- _CN_151706977_275000_CN_144077272_275000/LConn1
  東京北線_(Tōkyō_Kita_Sen)_CN_133137636_275000_CN_151706977_275000/RConn2 -- T_151706977__新野田変電所_(Shin_Noda_Hendensho)/RConn2 -- 新京葉線_CN_151706977_275000_CN_168852840_275000/RConn2 -- _CN_151706977_275000_CN_144077272_275000/LConn2
  東京北線_(Tōkyō_Kita_Sen)_CN_133137636_275000_CN_151706977_275000/RConn3 -- T_151706977__新野田変電所_(Shin_Noda_Hendensho)/RConn3 -- 新京葉線_CN_151706977_275000_CN_168852840_275000/RConn3 -- _CN_151706977_275000_CN_144077272_275000/LConn3
  西越谷線_(Nishi_Koshigaya_Sen)_CN_133137636_275000_CN_155411568_275000/RConn1 -- T_155411568__/LConn1 -- 西越谷線_(Nishi_Koshigaya_Sen)_CN_155411568_275000_CN_153521822_275000/LConn1
  西越谷線_(Nishi_Koshigaya_Sen)_CN_133137636_275000_CN_155411568_275000/RConn2 -- T_155411568__/LConn2 -- 西越谷線_(Nishi_Koshigaya_Sen)_CN_155411568_275000_CN_153521822_275000/LConn2
  西越谷線_(Nishi_Koshigaya_Sen)_CN_133137636_275000_CN_155411568_275000/RConn3 -- T_155411568__/LConn3 -- 西越谷線_(Nishi_Koshigaya_Sen)_CN_155411568_275000_CN_153521822_275000/LConn3
  T_145084773_275000_青梅変電所/LConn1 -- _CN_145084773_275000_CN_133644487_275000/LConn1
  T_145084773_275000_青梅変電所/LConn2 -- _CN_145084773_275000_CN_133644487_275000/LConn2
  T_145084773_275000_青梅変電所/LConn3 -- _CN_145084773_275000_CN_133644487_275000/LConn3
  T_133644487__/LConn1 -- _CN_145084773_275000_CN_133644487_275000/RConn1
  T_133644487__/LConn2 -- _CN_145084773_275000_CN_133644487_275000/RConn2
  T_133644487__/LConn3 -- _CN_145084773_275000_CN_133644487_275000/RConn3
  T_262597734__海部開閉所/LConn1 -- _CN_262597734_275000_CN_170793703_275000/RConn1
  T_262597734__海部開閉所/LConn2 -- _CN_262597734_275000_CN_170793703_275000/RConn2
  T_262597734__海部開閉所/LConn3 -- _CN_262597734_275000_CN_170793703_275000/RConn3
  _CN_87682157_275000_CN_128581912_275000/RConn1 -- T_87682157_275000_南川越変電所_(Minamikawagoe_Hendensho)/LConn1 -- _CN_87682157_275000_CN_159491797_275000/LConn1
  _CN_87682157_275000_CN_128581912_275000/RConn2 -- T_87682157_275000_南川越変電所_(Minamikawagoe_Hendensho)/LConn2 -- _CN_87682157_275000_CN_159491797_275000/LConn2
  _CN_87682157_275000_CN_128581912_275000/RConn3 -- T_87682157_275000_南川越変電所_(Minamikawagoe_Hendensho)/LConn3 -- _CN_87682157_275000_CN_159491797_275000/LConn3
  _CN_87682157_275000_CN_159491797_275000/RConn1 -- T_159491797_275000_南狭山変電所_(Minamisayama_Hendensho)/LConn1 -- _CN_159491797_275000_CN_136298957_275000/LConn1
  _CN_87682157_275000_CN_159491797_275000/RConn2 -- T_159491797_275000_南狭山変電所_(Minamisayama_Hendensho)/LConn2 -- _CN_159491797_275000_CN_136298957_275000/LConn2
  _CN_87682157_275000_CN_159491797_275000/RConn3 -- T_159491797_275000_南狭山変電所_(Minamisayama_Hendensho)/LConn3 -- _CN_159491797_275000_CN_136298957_275000/LConn3
  那珂線_(Naka_Sen)_CN_105291887_275000_CN_168839127_275000/LConn1 -- T_105291887_275000_那珂変電所_(Naka_Hendensho)/LConn1 -- _CN_105291887_275000_CN103827577/LConn1
  那珂線_(Naka_Sen)_CN_105291887_275000_CN_168839127_275000/LConn2 -- T_105291887_275000_那珂変電所_(Naka_Hendensho)/LConn2 -- _CN_105291887_275000_CN103827577/LConn2
  那珂線_(Naka_Sen)_CN_105291887_275000_CN_168839127_275000/LConn3 -- T_105291887_275000_那珂変電所_(Naka_Hendensho)/LConn3 -- _CN_105291887_275000_CN103827577/LConn3
  T_168839127__新茂木/RConn1 -- 那珂線_(Naka_Sen)_CN_105291887_275000_CN_168839127_275000/RConn1
  T_168839127__新茂木/RConn2 -- 那珂線_(Naka_Sen)_CN_105291887_275000_CN_168839127_275000/RConn2
  T_168839127__新茂木/RConn3 -- 那珂線_(Naka_Sen)_CN_105291887_275000_CN_168839127_275000/RConn3
  G_103827577_/RConn1 -- _CN_105291887_275000_CN103827577/RConn1
  G_103827577_/RConn2 -- _CN_105291887_275000_CN103827577/RConn2
  G_103827577_/RConn3 -- _CN_105291887_275000_CN103827577/RConn3
  T_153521822_275000_西越谷変電所_(Nishi_Koshigaya_Hendensho)/LConn1 -- 西越谷線_(Nishi_Koshigaya_Sen)_CN_155411568_275000_CN_153521822_275000/RConn1
  T_153521822_275000_西越谷変電所_(Nishi_Koshigaya_Hendensho)/LConn2 -- 西越谷線_(Nishi_Koshigaya_Sen)_CN_155411568_275000_CN_153521822_275000/RConn2
  T_153521822_275000_西越谷変電所_(Nishi_Koshigaya_Hendensho)/LConn3 -- 西越谷線_(Nishi_Koshigaya_Sen)_CN_155411568_275000_CN_153521822_275000/RConn3
  _CN_104530060_500000_CN_168839127_500000/RConn1 -- T_168839127__新茂木/LConn1 -- 福島幹線_CN_133135172_500000_CN_168839127_500000/LConn1 -- 福島幹線_CN_104391636_500000_CN_168839127_500000/LConn1
  _CN_104530060_500000_CN_168839127_500000/RConn2 -- T_168839127__新茂木/LConn2 -- 福島幹線_CN_133135172_500000_CN_168839127_500000/LConn2 -- 福島幹線_CN_104391636_500000_CN_168839127_500000/LConn2
  _CN_104530060_500000_CN_168839127_500000/RConn3 -- T_168839127__新茂木/LConn3 -- 福島幹線_CN_133135172_500000_CN_168839127_500000/LConn3 -- 福島幹線_CN_104391636_500000_CN_168839127_500000/LConn3
  T_315434358_500000_新岡部変電所/LConn1 -- _CN_104530060_500000_CN_315434358_500000/RConn1
  T_315434358_500000_新岡部変電所/LConn2 -- _CN_104530060_500000_CN_315434358_500000/RConn2
  T_315434358_500000_新岡部変電所/LConn3 -- _CN_104530060_500000_CN_315434358_500000/RConn3
  _CN_320438391_500000_CN_241822621_500000/LConn1 -- T_320438391_500000_/LConn1 -- _CN_320438391_500000_CN_169031921_500000/RConn1 -- _CN_320438391_500000_CN_110682956_500000/LConn1 -- _CN_320438391_500000_CN_320444665_500000/LConn1
  _CN_320438391_500000_CN_241822621_500000/LConn2 -- T_320438391_500000_/LConn2 -- _CN_320438391_500000_CN_169031921_500000/RConn2 -- _CN_320438391_500000_CN_110682956_500000/LConn2 -- _CN_320438391_500000_CN_320444665_500000/LConn2
  _CN_320438391_500000_CN_241822621_500000/LConn3 -- T_320438391_500000_/LConn3 -- _CN_320438391_500000_CN_169031921_500000/RConn3 -- _CN_320438391_500000_CN_110682956_500000/LConn3 -- _CN_320438391_500000_CN_320444665_500000/LConn3
  _CN_320438391_500000_CN_241822621_500000/RConn1 -- T_241822621_500000_/LConn1 -- _CN_242253537_500000_CN_241822621_500000/LConn1 -- _CN_241822621_500000_CN_241822631_500000/LConn1
  _CN_320438391_500000_CN_241822621_500000/RConn2 -- T_241822621_500000_/LConn2 -- _CN_242253537_500000_CN_241822621_500000/LConn2 -- _CN_241822621_500000_CN_241822631_500000/LConn2
  _CN_320438391_500000_CN_241822621_500000/RConn3 -- T_241822621_500000_/LConn3 -- _CN_242253537_500000_CN_241822621_500000/LConn3 -- _CN_241822621_500000_CN_241822631_500000/LConn3
  _CN_320438391_500000_CN_110682956_500000/RConn1 -- T_110682956_500000_猪名川変電所/LConn1 -- _CN_170605907_500000_CN_110682956_500000/LConn1
  _CN_320438391_500000_CN_110682956_500000/RConn2 -- T_110682956_500000_猪名川変電所/LConn2 -- _CN_170605907_500000_CN_110682956_500000/LConn2
  _CN_320438391_500000_CN_110682956_500000/RConn3 -- T_110682956_500000_猪名川変電所/LConn3 -- _CN_170605907_500000_CN_110682956_500000/LConn3
  T_320444665_500000_/LConn1 -- _CN_320438391_500000_CN_320444665_500000/RConn1
  T_320444665_500000_/LConn2 -- _CN_320438391_500000_CN_320444665_500000/RConn2
  T_320444665_500000_/LConn3 -- _CN_320438391_500000_CN_320444665_500000/RConn3
  T_179417733_275000_/LConn1 -- _CN_179417733_275000_CN180359744/LConn1
  T_179417733_275000_/LConn2 -- _CN_179417733_275000_CN180359744/LConn2
  T_179417733_275000_/LConn3 -- _CN_179417733_275000_CN180359744/LConn3
  G_180359744_知多火力発電所/RConn1 -- _CN_179417733_275000_CN180359744/RConn1
  G_180359744_知多火力発電所/RConn2 -- _CN_179417733_275000_CN180359744/RConn2
  G_180359744_知多火力発電所/RConn3 -- _CN_179417733_275000_CN180359744/RConn3
  T_161948515_275000_西濃変電所_(Seinō_Hendensho)/LConn1 -- _CN_161946849_275000_CN_161948515_275000/RConn1
  T_161948515_275000_西濃変電所_(Seinō_Hendensho)/LConn2 -- _CN_161946849_275000_CN_161948515_275000/RConn2
  T_161948515_275000_西濃変電所_(Seinō_Hendensho)/LConn3 -- _CN_161946849_275000_CN_161948515_275000/RConn3
  _CN_161946849_275000_CN210658603/RConn1 -- G_210658603_高根第一水力発電所/RConn1 -- _CN_315662816_275000_CN210658603/LConn1
  _CN_161946849_275000_CN210658603/RConn2 -- G_210658603_高根第一水力発電所/RConn2 -- _CN_315662816_275000_CN210658603/LConn2
  _CN_161946849_275000_CN210658603/RConn3 -- G_210658603_高根第一水力発電所/RConn3 -- _CN_315662816_275000_CN210658603/LConn3
  T_315461259_500000_/LConn1 -- 富津火力線_CN_315461259_500000_CN_315461272_500000/LConn1
  T_315461259_500000_/LConn2 -- 富津火力線_CN_315461259_500000_CN_315461272_500000/LConn2
  T_315461259_500000_/LConn3 -- 富津火力線_CN_315461259_500000_CN_315461272_500000/LConn3
  富津火力線_CN_315461259_500000_CN_315461272_500000/RConn1 -- T_315461272_500000_新木更津変電所/LConn1 -- _CN_315461272_500000_CN_105298089_500000/LConn1
  富津火力線_CN_315461259_500000_CN_315461272_500000/RConn2 -- T_315461272_500000_新木更津変電所/LConn2 -- _CN_315461272_500000_CN_105298089_500000/LConn2
  富津火力線_CN_315461259_500000_CN_315461272_500000/RConn3 -- T_315461272_500000_新木更津変電所/LConn3 -- _CN_315461272_500000_CN_105298089_500000/LConn3
  T_170247308_275000_三河変電所/LConn1 -- 湖西三河線_CN_170247308_275000_CN_170260165_275000/LConn1
  T_170247308_275000_三河変電所/LConn2 -- 湖西三河線_CN_170247308_275000_CN_170260165_275000/LConn2
  T_170247308_275000_三河変電所/LConn3 -- 湖西三河線_CN_170247308_275000_CN_170260165_275000/LConn3
  T_170260165_275000_中部電力湖西変電所/LConn1 -- 湖西三河線_CN_170247308_275000_CN_170260165_275000/RConn1
  T_170260165_275000_中部電力湖西変電所/LConn2 -- 湖西三河線_CN_170247308_275000_CN_170260165_275000/RConn2
  T_170260165_275000_中部電力湖西変電所/LConn3 -- 湖西三河線_CN_170247308_275000_CN_170260165_275000/RConn3
  T_128581912_500000;275000;66000_新坂戸変電所/LConn1 -- 新坂戸線_CN_128581912_500000_CN_133641619_500000/LConn1
  T_128581912_500000;275000;66000_新坂戸変電所/LConn2 -- 新坂戸線_CN_128581912_500000_CN_133641619_500000/LConn2
  T_128581912_500000;275000;66000_新坂戸変電所/LConn3 -- 新坂戸線_CN_128581912_500000_CN_133641619_500000/LConn3
  新坂戸線_CN_128581912_500000_CN_133641619_500000/RConn1 -- T_133641619_500000_新所沢変電所_(Shin_Tokorozawa_Hendensho)/LConn1 -- 新所沢線_(Shin_Tokorozawa_Sen)_CN_133641619_500000_CN_145079972_500000/RConn1 -- 新古河線_(Shin_Koga_Sen)_CN_133135172_500000_CN_133641619_500000/LConn1
  新坂戸線_CN_128581912_500000_CN_133641619_500000/RConn2 -- T_133641619_500000_新所沢変電所_(Shin_Tokorozawa_Hendensho)/LConn2 -- 新所沢線_(Shin_Tokorozawa_Sen)_CN_133641619_500000_CN_145079972_500000/RConn2 -- 新古河線_(Shin_Koga_Sen)_CN_133135172_500000_CN_133641619_500000/LConn2
  新坂戸線_CN_128581912_500000_CN_133641619_500000/RConn3 -- T_133641619_500000_新所沢変電所_(Shin_Tokorozawa_Hendensho)/LConn3 -- 新所沢線_(Shin_Tokorozawa_Sen)_CN_133641619_500000_CN_145079972_500000/RConn3 -- 新古河線_(Shin_Koga_Sen)_CN_133135172_500000_CN_133641619_500000/LConn3
  T_170247314_275000_額田開閉所/LConn1 -- _CN_170247314_275000_CN_170247359_275000/RConn1
  T_170247314_275000_額田開閉所/LConn2 -- _CN_170247314_275000_CN_170247359_275000/RConn2
  T_170247314_275000_額田開閉所/LConn3 -- _CN_170247314_275000_CN_170247359_275000/RConn3
  _CN_315608215_500000_CN_169249243_500000/LConn1 -- T_315608215_500000_/LConn1 -- _CN_315608215_500000_CN_169249247_500000/LConn1 -- 志賀中能登線_CN_315608215_500000_CN255763556/LConn1
  _CN_315608215_500000_CN_169249243_500000/LConn2 -- T_315608215_500000_/LConn2 -- _CN_315608215_500000_CN_169249247_500000/LConn2 -- 志賀中能登線_CN_315608215_500000_CN255763556/LConn2
  _CN_315608215_500000_CN_169249243_500000/LConn3 -- T_315608215_500000_/LConn3 -- _CN_315608215_500000_CN_169249247_500000/LConn3 -- 志賀中能登線_CN_315608215_500000_CN255763556/LConn3
  _CN_315608215_500000_CN_169249243_500000/RConn1 -- T_169249243_500000_南福光変電所/LConn1 -- 加賀福光線_CN_169249243_500000_CN_169249247_500000/LConn1
  _CN_315608215_500000_CN_169249243_500000/RConn2 -- T_169249243_500000_南福光変電所/LConn2 -- 加賀福光線_CN_169249243_500000_CN_169249247_500000/LConn2
  _CN_315608215_500000_CN_169249243_500000/RConn3 -- T_169249243_500000_南福光変電所/LConn3 -- 加賀福光線_CN_169249243_500000_CN_169249247_500000/LConn3
  _CN_315608215_500000_CN_169249247_500000/RConn1 -- T_169249247_500000_加賀変電所/LConn1 -- 加賀福光線_CN_169249243_500000_CN_169249247_500000/RConn1
  _CN_315608215_500000_CN_169249247_500000/RConn2 -- T_169249247_500000_加賀変電所/LConn2 -- 加賀福光線_CN_169249243_500000_CN_169249247_500000/RConn2
  _CN_315608215_500000_CN_169249247_500000/RConn3 -- T_169249247_500000_加賀変電所/LConn3 -- 加賀福光線_CN_169249243_500000_CN_169249247_500000/RConn3
  G_255763556_志賀原子力発電所/RConn1 -- 志賀中能登線_CN_315608215_500000_CN255763556/RConn1
  G_255763556_志賀原子力発電所/RConn2 -- 志賀中能登線_CN_315608215_500000_CN255763556/RConn2
  G_255763556_志賀原子力発電所/RConn3 -- 志賀中能登線_CN_315608215_500000_CN255763556/RConn3
  _CN_315461272_500000_CN_105298089_500000/RConn1 -- T_105298089_500000_新佐原変電所/LConn1 -- 新佐原線_CN_132913106_500000_CN_105298089_500000/LConn1 -- _CN_105298089_500000_CN_168727982_500000/LConn1
  _CN_315461272_500000_CN_105298089_500000/RConn2 -- T_105298089_500000_新佐原変電所/LConn2 -- 新佐原線_CN_132913106_500000_CN_105298089_500000/LConn2 -- _CN_105298089_500000_CN_168727982_500000/LConn2
  _CN_315461272_500000_CN_105298089_500000/RConn3 -- T_105298089_500000_新佐原変電所/LConn3 -- 新佐原線_CN_132913106_500000_CN_105298089_500000/LConn3 -- _CN_105298089_500000_CN_168727982_500000/LConn3
  _CN_302164677_275000_CN_316727625_275000/LConn1 -- T_302164677__秋田変電所/LConn1 -- _CN_302164677_275000_CN_302164679_275000/LConn1
  _CN_302164677_275000_CN_316727625_275000/LConn2 -- T_302164677__秋田変電所/LConn2 -- _CN_302164677_275000_CN_302164679_275000/LConn2
  _CN_302164677_275000_CN_316727625_275000/LConn3 -- T_302164677__秋田変電所/LConn3 -- _CN_302164677_275000_CN_302164679_275000/LConn3
  T_316727625_275000_/LConn1 -- _CN_302164677_275000_CN_316727625_275000/RConn1
  T_316727625_275000_/LConn2 -- _CN_302164677_275000_CN_316727625_275000/RConn2
  T_316727625_275000_/LConn3 -- _CN_302164677_275000_CN_316727625_275000/RConn3
  _CN_302164677_275000_CN_302164679_275000/RConn1 -- T_302164679_275000_能代変電所/LConn1 -- _CN_302164679_275000_CN_316581637_275000/LConn1
  _CN_302164677_275000_CN_302164679_275000/RConn2 -- T_302164679_275000_能代変電所/LConn2 -- _CN_302164679_275000_CN_316581637_275000/LConn2
  _CN_302164677_275000_CN_302164679_275000/RConn3 -- T_302164679_275000_能代変電所/LConn3 -- _CN_302164679_275000_CN_316581637_275000/LConn3
  _CN_170974371_500000_CN_241828221_500000/RConn1 -- T_241828221_500000_新岡山変電所_(Shin_Okayama_Hendensho)/LConn1 -- _CN_241828221_500000_CN_241822623_500000/LConn1 -- _CN_242103481_500000_CN_241828221_500000/LConn1
  _CN_170974371_500000_CN_241828221_500000/RConn2 -- T_241828221_500000_新岡山変電所_(Shin_Okayama_Hendensho)/LConn2 -- _CN_241828221_500000_CN_241822623_500000/LConn2 -- _CN_242103481_500000_CN_241828221_500000/LConn2
  _CN_170974371_500000_CN_241828221_500000/RConn3 -- T_241828221_500000_新岡山変電所_(Shin_Okayama_Hendensho)/LConn3 -- _CN_241828221_500000_CN_241822623_500000/LConn3 -- _CN_242103481_500000_CN_241828221_500000/LConn3
  _CN_317416612_500000_CN_242103481_500000/RConn1 -- T_242103481_500000_日野変電所/LConn1 -- _CN_242253537_500000_CN_242103481_500000/LConn1 -- _CN_242103481_500000_CN_241828221_500000/RConn1 -- _CN_317511904_500000_CN_242103481_500000/LConn1
  _CN_317416612_500000_CN_242103481_500000/RConn2 -- T_242103481_500000_日野変電所/LConn2 -- _CN_242253537_500000_CN_242103481_500000/LConn2 -- _CN_242103481_500000_CN_241828221_500000/RConn2 -- _CN_317511904_500000_CN_242103481_500000/LConn2
  _CN_317416612_500000_CN_242103481_500000/RConn3 -- T_242103481_500000_日野変電所/LConn3 -- _CN_242253537_500000_CN_242103481_500000/LConn3 -- _CN_242103481_500000_CN_241828221_500000/RConn3 -- _CN_317511904_500000_CN_242103481_500000/LConn3
  _CN_317416612_500000_CN_204258596_500000/RConn1 -- T_204258596_500000_/LConn1 -- _CN_242253500_500000_CN_204258596_500000/RConn1 -- 関門連系線_CN_204258596_500000_CN_187988970_500000/RConn1
  _CN_317416612_500000_CN_204258596_500000/RConn2 -- T_204258596_500000_/LConn2 -- _CN_242253500_500000_CN_204258596_500000/RConn2 -- 関門連系線_CN_204258596_500000_CN_187988970_500000/RConn2
  _CN_317416612_500000_CN_204258596_500000/RConn3 -- T_204258596_500000_/LConn3 -- _CN_242253500_500000_CN_204258596_500000/RConn3 -- 関門連系線_CN_204258596_500000_CN_187988970_500000/RConn3
  T_315757225_275000_/LConn1 -- _CN_315757225_275000_CN_256682313_275000/RConn1
  T_315757225_275000_/LConn2 -- _CN_315757225_275000_CN_256682313_275000/RConn2
  T_315757225_275000_/LConn3 -- _CN_315757225_275000_CN_256682313_275000/RConn3
  T_316581637_275000_青森変電所/LConn1 -- _CN_302164679_275000_CN_316581637_275000/RConn1
  T_316581637_275000_青森変電所/LConn2 -- _CN_302164679_275000_CN_316581637_275000/RConn2
  T_316581637_275000_青森変電所/LConn3 -- _CN_302164679_275000_CN_316581637_275000/RConn3
  _CN_87538349_500000_CN_171066843_500000/LConn1 -- T_87538349_500000_讃岐変電所/LConn1 -- _CN_87538349_500000_CN_102958903_500000/LConn1
  _CN_87538349_500000_CN_171066843_500000/LConn2 -- T_87538349_500000_讃岐変電所/LConn2 -- _CN_87538349_500000_CN_102958903_500000/LConn2
  _CN_87538349_500000_CN_171066843_500000/LConn3 -- T_87538349_500000_讃岐変電所/LConn3 -- _CN_87538349_500000_CN_102958903_500000/LConn3
  T_171066843_500000_四国電力東予変電所/LConn1 -- _CN_87538349_500000_CN_171066843_500000/RConn1
  T_171066843_500000_四国電力東予変電所/LConn2 -- _CN_87538349_500000_CN_171066843_500000/RConn2
  T_171066843_500000_四国電力東予変電所/LConn3 -- _CN_87538349_500000_CN_171066843_500000/RConn3
  T_102958903_500000_/LConn1 -- _CN_87538349_500000_CN_102958903_500000/RConn1
  T_102958903_500000_/LConn2 -- _CN_87538349_500000_CN_102958903_500000/RConn2
  T_102958903_500000_/LConn3 -- _CN_87538349_500000_CN_102958903_500000/RConn3
  _CN_242253497_275000_CN_185032690_275000/LConn1 -- T_242253497_275000_姫路変電所_(Himeji_Hendensho)/LConn1 -- _CN_242253497_275000_CN_241822631_275000/LConn1
  _CN_242253497_275000_CN_185032690_275000/LConn2 -- T_242253497_275000_姫路変電所_(Himeji_Hendensho)/LConn2 -- _CN_242253497_275000_CN_241822631_275000/LConn2
  _CN_242253497_275000_CN_185032690_275000/LConn3 -- T_242253497_275000_姫路変電所_(Himeji_Hendensho)/LConn3 -- _CN_242253497_275000_CN_241822631_275000/LConn3
  _CN_242253497_275000_CN_185032690_275000/RConn1 -- T_185032690_275000_西神戸変電所/LConn1 -- _CN_185032690_275000_CN110340505/LConn1
  _CN_242253497_275000_CN_185032690_275000/RConn2 -- T_185032690_275000_西神戸変電所/LConn2 -- _CN_185032690_275000_CN110340505/LConn2
  _CN_242253497_275000_CN_185032690_275000/RConn3 -- T_185032690_275000_西神戸変電所/LConn3 -- _CN_185032690_275000_CN110340505/LConn3
  _CN_242253497_275000_CN_241822631_275000/RConn1 -- T_241822631__/RConn1 -- _CN_241822631_275000_CN242706111/LConn1
  _CN_242253497_275000_CN_241822631_275000/RConn2 -- T_241822631__/RConn2 -- _CN_241822631_275000_CN242706111/LConn2
  _CN_242253497_275000_CN_241822631_275000/RConn3 -- T_241822631__/RConn3 -- _CN_241822631_275000_CN242706111/LConn3
  T_160374974_275000;77000_北葛城変電所_(Kita_Katsuragi_Hendensho)/LConn1 -- 北葛城線_(Kita_Katsuragi_Sen)_CN_160374974_275000_CN_109834508_275000/RConn1
  T_160374974_275000;77000_北葛城変電所_(Kita_Katsuragi_Hendensho)/LConn2 -- 北葛城線_(Kita_Katsuragi_Sen)_CN_160374974_275000_CN_109834508_275000/RConn2
  T_160374974_275000;77000_北葛城変電所_(Kita_Katsuragi_Hendensho)/LConn3 -- 北葛城線_(Kita_Katsuragi_Sen)_CN_160374974_275000_CN_109834508_275000/RConn3
  T_216956620_500000_/LConn1 -- 小丸川幹線_CN_216956620_500000_CN216953915/LConn1
  T_216956620_500000_/LConn2 -- 小丸川幹線_CN_216956620_500000_CN216953915/LConn2
  T_216956620_500000_/LConn3 -- 小丸川幹線_CN_216956620_500000_CN216953915/LConn3
  G_216953915_/RConn1 -- 小丸川幹線_CN_216956620_500000_CN216953915/RConn1
  G_216953915_/RConn2 -- 小丸川幹線_CN_216956620_500000_CN216953915/RConn2
  G_216953915_/RConn3 -- 小丸川幹線_CN_216956620_500000_CN216953915/RConn3
  T_159191758_275000_北松本変電所/LConn1 -- _CN_159191758_275000_CN_211258348_275000/LConn1
  T_159191758_275000_北松本変電所/LConn2 -- _CN_159191758_275000_CN_211258348_275000/LConn2
  T_159191758_275000_北松本変電所/LConn3 -- _CN_159191758_275000_CN_211258348_275000/LConn3
  _CN_159191758_275000_CN_211258348_275000/RConn1 -- T_211258348_275000_東信変電所/LConn1 -- _CN_199544541_275000_CN_211258348_275000/LConn1
  _CN_159191758_275000_CN_211258348_275000/RConn2 -- T_211258348_275000_東信変電所/LConn2 -- _CN_199544541_275000_CN_211258348_275000/LConn2
  _CN_159191758_275000_CN_211258348_275000/RConn3 -- T_211258348_275000_東信変電所/LConn3 -- _CN_199544541_275000_CN_211258348_275000/LConn3
  _CN_253566674_500000_CN_104391636_500000/LConn1 -- T_253566674__/LConn1 -- _CN_253566674_500000_CN_156208858_500000/LConn1
  _CN_253566674_500000_CN_104391636_500000/LConn2 -- T_253566674__/LConn2 -- _CN_253566674_500000_CN_156208858_500000/LConn2
  _CN_253566674_500000_CN_104391636_500000/LConn3 -- T_253566674__/LConn3 -- _CN_253566674_500000_CN_156208858_500000/LConn3
  _CN_253566674_500000_CN_104391636_500000/RConn1 -- T_104391636_500000_新いわき/LConn1 -- _CN_132913106_500000_CN_104391636_500000/LConn1 -- 福島東幹線2_CN_106309481_500000_CN_104391636_500000/RConn1 -- 福島幹線_CN_104391636_500000_CN_168839127_500000/RConn1
  _CN_253566674_500000_CN_104391636_500000/RConn2 -- T_104391636_500000_新いわき/LConn2 -- _CN_132913106_500000_CN_104391636_500000/LConn2 -- 福島東幹線2_CN_106309481_500000_CN_104391636_500000/RConn2 -- 福島幹線_CN_104391636_500000_CN_168839127_500000/RConn2
  _CN_253566674_500000_CN_104391636_500000/RConn3 -- T_104391636_500000_新いわき/LConn3 -- _CN_132913106_500000_CN_104391636_500000/LConn3 -- 福島東幹線2_CN_106309481_500000_CN_104391636_500000/RConn3 -- 福島幹線_CN_104391636_500000_CN_168839127_500000/RConn3
  T_156208858_500000_南相馬変電所/LConn1 -- _CN_253566674_500000_CN_156208858_500000/RConn1
  T_156208858_500000_南相馬変電所/LConn2 -- _CN_253566674_500000_CN_156208858_500000/RConn2
  T_156208858_500000_南相馬変電所/LConn3 -- _CN_253566674_500000_CN_156208858_500000/RConn3
  T_136298957__新座変電所/LConn1 -- _CN_159491797_275000_CN_136298957_275000/RConn1
  T_136298957__新座変電所/LConn2 -- _CN_159491797_275000_CN_136298957_275000/RConn2
  T_136298957__新座変電所/LConn3 -- _CN_159491797_275000_CN_136298957_275000/RConn3
  _CN_169963227_500000_CN_169963236_500000/LConn1 -- T_169963227_500000_新榛名/LConn1 -- 新榛名線_CN_169963227_500000_CN_195615141_500000/LConn1
  _CN_169963227_500000_CN_169963236_500000/LConn2 -- T_169963227_500000_新榛名/LConn2 -- 新榛名線_CN_169963227_500000_CN_195615141_500000/LConn2
  _CN_169963227_500000_CN_169963236_500000/LConn3 -- T_169963227_500000_新榛名/LConn3 -- 新榛名線_CN_169963227_500000_CN_195615141_500000/LConn3
  _CN_169963227_500000_CN_169963236_500000/RConn1 -- T_169963236__/LConn1 -- 新吾妻線_CN_169963236_500000_CN_66098469_500000/RConn1
  _CN_169963227_500000_CN_169963236_500000/RConn2 -- T_169963236__/LConn2 -- 新吾妻線_CN_169963236_500000_CN_66098469_500000/RConn2
  _CN_169963227_500000_CN_169963236_500000/RConn3 -- T_169963236__/LConn3 -- 新吾妻線_CN_169963236_500000_CN_66098469_500000/RConn3
  新榛名線_CN_169963227_500000_CN_195615141_500000/RConn1 -- T_195615141_500000_/LConn1 -- _CN_195615141_500000_CN_145079972_500000/RConn1 -- _CN_195615141_500000_CN_315662839_500000/LConn1
  新榛名線_CN_169963227_500000_CN_195615141_500000/RConn2 -- T_195615141_500000_/LConn2 -- _CN_195615141_500000_CN_145079972_500000/RConn2 -- _CN_195615141_500000_CN_315662839_500000/LConn2
  新榛名線_CN_169963227_500000_CN_195615141_500000/RConn3 -- T_195615141_500000_/LConn3 -- _CN_195615141_500000_CN_145079972_500000/RConn3 -- _CN_195615141_500000_CN_315662839_500000/LConn3
  T_199544541_275000_新北信変電所/LConn1 -- _CN_199544541_275000_CN_211258348_275000/RConn1
  T_199544541_275000_新北信変電所/LConn2 -- _CN_199544541_275000_CN_211258348_275000/RConn2
  T_199544541_275000_新北信変電所/LConn3 -- _CN_199544541_275000_CN_211258348_275000/RConn3
  T_317511904_500000_北松江変電所/LConn1 -- _CN_317511904_500000_CN_242103481_500000/RConn1
  T_317511904_500000_北松江変電所/LConn2 -- _CN_317511904_500000_CN_242103481_500000/RConn2
  T_317511904_500000_北松江変電所/LConn3 -- _CN_317511904_500000_CN_242103481_500000/RConn3
  _CN_242253537_500000_CN_242103481_500000/RConn1 -- T_242253537__/LConn1 -- _CN_242253537_500000_CN_241822621_500000/RConn1
  _CN_242253537_500000_CN_242103481_500000/RConn2 -- T_242253537__/LConn2 -- _CN_242253537_500000_CN_241822621_500000/RConn2
  _CN_242253537_500000_CN_242103481_500000/RConn3 -- T_242253537__/LConn3 -- _CN_242253537_500000_CN_241822621_500000/RConn3
  T_210765350__花見川変電所_(Hanamigawa_Hendensho)/LConn1 -- 花見川線_CN_210765350_275000_CN_211241774_275000/LConn1
  T_210765350__花見川変電所_(Hanamigawa_Hendensho)/LConn2 -- 花見川線_CN_210765350_275000_CN_211241774_275000/LConn2
  T_210765350__花見川変電所_(Hanamigawa_Hendensho)/LConn3 -- 花見川線_CN_210765350_275000_CN_211241774_275000/LConn3
  T_211241774__/LConn1 -- 花見川線_CN_210765350_275000_CN_211241774_275000/RConn1
  T_211241774__/LConn2 -- 花見川線_CN_210765350_275000_CN_211241774_275000/RConn2
  T_211241774__/LConn3 -- 花見川線_CN_210765350_275000_CN_211241774_275000/RConn3
  _CN_170793702_275000_CN_170793703_275000/RConn1 -- T_170793702_275000_西名古屋/LConn1 -- _CN_170793702_275000_CN180359727/LConn1
  _CN_170793702_275000_CN_170793703_275000/RConn2 -- T_170793702_275000_西名古屋/LConn2 -- _CN_170793702_275000_CN180359727/LConn2
  _CN_170793702_275000_CN_170793703_275000/RConn3 -- T_170793702_275000_西名古屋/LConn3 -- _CN_170793702_275000_CN180359727/LConn3
  G_180359727_川越火力発電所/RConn1 -- _CN_170793702_275000_CN180359727/RConn1
  G_180359727_川越火力発電所/RConn2 -- _CN_170793702_275000_CN180359727/RConn2
  G_180359727_川越火力発電所/RConn3 -- _CN_170793702_275000_CN180359727/RConn3
  _CN_179863079_275000_CN_256894928_275000/LConn1 -- T_179863079_275000_/LConn1 -- 道央北幹線_CN_179863079_275000_CN_168524732_275000/LConn1
  _CN_179863079_275000_CN_256894928_275000/LConn2 -- T_179863079_275000_/LConn2 -- 道央北幹線_CN_179863079_275000_CN_168524732_275000/LConn2
  _CN_179863079_275000_CN_256894928_275000/LConn3 -- T_179863079_275000_/LConn3 -- 道央北幹線_CN_179863079_275000_CN_168524732_275000/LConn3
  T_256894928__/LConn1 -- _CN_179863079_275000_CN_256894928_275000/RConn1
  T_256894928__/LConn2 -- _CN_179863079_275000_CN_256894928_275000/RConn2
  T_256894928__/LConn3 -- _CN_179863079_275000_CN_256894928_275000/RConn3
  T_168524732__/LConn1 -- 道央北幹線_CN_179863079_275000_CN_168524732_275000/RConn1
  T_168524732__/LConn2 -- 道央北幹線_CN_179863079_275000_CN_168524732_275000/RConn2
  T_168524732__/LConn3 -- 道央北幹線_CN_179863079_275000_CN_168524732_275000/RConn3
  T_242103532_500000_/LConn1 -- _CN_242103532_500000_CN_241822623_500000/LConn1
  T_242103532_500000_/LConn2 -- _CN_242103532_500000_CN_241822623_500000/LConn2
  T_242103532_500000_/LConn3 -- _CN_242103532_500000_CN_241822623_500000/LConn3
  _CN_242103532_500000_CN_241822623_500000/RConn1 -- T_241822623_500000;220000;110000_/LConn1 -- _CN_241822623_500000_CN_241822631_500000/LConn1 -- _CN_241828221_500000_CN_241822623_500000/RConn1
  _CN_242103532_500000_CN_241822623_500000/RConn2 -- T_241822623_500000;220000;110000_/LConn2 -- _CN_241822623_500000_CN_241822631_500000/LConn2 -- _CN_241828221_500000_CN_241822623_500000/RConn2
  _CN_242103532_500000_CN_241822623_500000/RConn3 -- T_241822623_500000;220000;110000_/LConn3 -- _CN_241822623_500000_CN_241822631_500000/LConn3 -- _CN_241828221_500000_CN_241822623_500000/RConn3
  京浜線1;2号線_CN_128364781_275000_CN_47110637_275000/RConn1 -- T_47110637_275000_西東京変電所/LConn1 -- 東京西線_CN_145080115_275000_CN_47110637_275000/LConn1 -- 只見幹線_CN_153760214_275000_CN_47110637_275000/LConn1
  京浜線1;2号線_CN_128364781_275000_CN_47110637_275000/RConn2 -- T_47110637_275000_西東京変電所/LConn2 -- 東京西線_CN_145080115_275000_CN_47110637_275000/LConn2 -- 只見幹線_CN_153760214_275000_CN_47110637_275000/LConn2
  京浜線1;2号線_CN_128364781_275000_CN_47110637_275000/RConn3 -- T_47110637_275000_西東京変電所/LConn3 -- 東京西線_CN_145080115_275000_CN_47110637_275000/LConn3 -- 只見幹線_CN_153760214_275000_CN_47110637_275000/LConn3
  T_169031922__/LConn1 -- _CN_169031922_500000_CN_169031998_500000/LConn1
  T_169031922__/LConn2 -- _CN_169031922_500000_CN_169031998_500000/LConn2
  T_169031922__/LConn3 -- _CN_169031922_500000_CN_169031998_500000/LConn3
  _CN_169031922_500000_CN_169031998_500000/RConn1 -- T_169031998__/LConn1 -- _CN_169031998_500000_CN_161870227_500000/RConn1 -- _CN_169031998_500000_CN_109850439_500000/LConn1
  _CN_169031922_500000_CN_169031998_500000/RConn2 -- T_169031998__/LConn2 -- _CN_169031998_500000_CN_161870227_500000/RConn2 -- _CN_169031998_500000_CN_109850439_500000/LConn2
  _CN_169031922_500000_CN_169031998_500000/RConn3 -- T_169031998__/LConn3 -- _CN_169031998_500000_CN_161870227_500000/RConn3 -- _CN_169031998_500000_CN_109850439_500000/LConn3
  T_104375141_275000_須賀川変電所_(Sukagawa_Hendensho)/LConn1 -- _CN_104375141_275000_CN_107262429_275000/LConn1
  T_104375141_275000_須賀川変電所_(Sukagawa_Hendensho)/LConn2 -- _CN_104375141_275000_CN_107262429_275000/LConn2
  T_104375141_275000_須賀川変電所_(Sukagawa_Hendensho)/LConn3 -- _CN_104375141_275000_CN_107262429_275000/LConn3
  _CN_104375141_275000_CN_107262429_275000/RConn1 -- T_107262429_275000_福島変電所/LConn1 -- _CN_316459359_275000_CN_107262429_275000/LConn1 -- _CN_250430935_275000_CN_107262429_275000/RConn1
  _CN_104375141_275000_CN_107262429_275000/RConn2 -- T_107262429_275000_福島変電所/LConn2 -- _CN_316459359_275000_CN_107262429_275000/LConn2 -- _CN_250430935_275000_CN_107262429_275000/RConn2
  _CN_104375141_275000_CN_107262429_275000/RConn3 -- T_107262429_275000_福島変電所/LConn3 -- _CN_316459359_275000_CN_107262429_275000/LConn3 -- _CN_250430935_275000_CN_107262429_275000/RConn3
  T_250540807_500000_東群馬変電所_(Higashi_Gunma_Substation)/LConn1 -- 東群馬幹線_CN_250540807_500000_CN_66098469_500000/RConn1
  T_250540807_500000_東群馬変電所_(Higashi_Gunma_Substation)/LConn2 -- 東群馬幹線_CN_250540807_500000_CN_66098469_500000/RConn2
  T_250540807_500000_東群馬変電所_(Higashi_Gunma_Substation)/LConn3 -- 東群馬幹線_CN_250540807_500000_CN_66098469_500000/RConn3
  G_354115662_沼沢発電所/RConn1 -- _CN_250430935_275000_CN354115662/RConn1
  G_354115662_沼沢発電所/RConn2 -- _CN_250430935_275000_CN354115662/RConn2
  G_354115662_沼沢発電所/RConn3 -- _CN_250430935_275000_CN354115662/RConn3
  T_291678103_275000_紀の川変電所_(Kinokawa_Hendensho)/LConn1 -- 金剛線_(Kongō_sen)_CN_109834508_275000_CN_291678103_275000/RConn1
  T_291678103_275000_紀の川変電所_(Kinokawa_Hendensho)/LConn2 -- 金剛線_(Kongō_sen)_CN_109834508_275000_CN_291678103_275000/RConn2
  T_291678103_275000_紀の川変電所_(Kinokawa_Hendensho)/LConn3 -- 金剛線_(Kongō_sen)_CN_109834508_275000_CN_291678103_275000/RConn3
  T_151379730_500000_房総変電所_(Bōsō_Hendensho)/LConn1 -- 房総線_CN_151379730_500000_CN_168727982_500000/LConn1
  T_151379730_500000_房総変電所_(Bōsō_Hendensho)/LConn2 -- 房総線_CN_151379730_500000_CN_168727982_500000/LConn2
  T_151379730_500000_房総変電所_(Bōsō_Hendensho)/LConn3 -- 房総線_CN_151379730_500000_CN_168727982_500000/LConn3
  房総線_CN_151379730_500000_CN_168727982_500000/RConn1 -- T_168727982_500000_新京葉変電所/LConn1 -- _CN_105298089_500000_CN_168727982_500000/RConn1 -- 新京葉線_CN_133135172_500000_CN_168727982_500000/LConn1
  房総線_CN_151379730_500000_CN_168727982_500000/RConn2 -- T_168727982_500000_新京葉変電所/LConn2 -- _CN_105298089_500000_CN_168727982_500000/RConn2 -- 新京葉線_CN_133135172_500000_CN_168727982_500000/LConn2
  房総線_CN_151379730_500000_CN_168727982_500000/RConn3 -- T_168727982_500000_新京葉変電所/LConn3 -- _CN_105298089_500000_CN_168727982_500000/RConn3 -- 新京葉線_CN_133135172_500000_CN_168727982_500000/LConn3
  G_215429864_川内原子力発電所/RConn1 -- _CN_215451416_500000_CN215429864/RConn1
  G_215429864_川内原子力発電所/RConn2 -- _CN_215451416_500000_CN215429864/RConn2
  G_215429864_川内原子力発電所/RConn3 -- _CN_215451416_500000_CN215429864/RConn3
  T_325868333_275000_/LConn1 -- _CN_325868333_275000_CN_110682951_275000/LConn1
  T_325868333_275000_/LConn2 -- _CN_325868333_275000_CN_110682951_275000/LConn2
  T_325868333_275000_/LConn3 -- _CN_325868333_275000_CN_110682951_275000/LConn3
  _CN_325868333_275000_CN_110682951_275000/RConn1 -- T_110682951_275000_宝塚開閉所_(Takarazuka_Kaiheisho)/LConn1 -- _CN_110682951_275000_CN_110682955_275000/LConn1
  _CN_325868333_275000_CN_110682951_275000/RConn2 -- T_110682951_275000_宝塚開閉所_(Takarazuka_Kaiheisho)/LConn2 -- _CN_110682951_275000_CN_110682955_275000/LConn2
  _CN_325868333_275000_CN_110682951_275000/RConn3 -- T_110682951_275000_宝塚開閉所_(Takarazuka_Kaiheisho)/LConn3 -- _CN_110682951_275000_CN_110682955_275000/LConn3
  T_145080115_275000_/LConn1 -- 東京西線_CN_145080115_275000_CN_47110637_275000/RConn1
  T_145080115_275000_/LConn2 -- 東京西線_CN_145080115_275000_CN_47110637_275000/RConn2
  T_145080115_275000_/LConn3 -- 東京西線_CN_145080115_275000_CN_47110637_275000/RConn3
  T_168903220_275000_/LConn1 -- _CN_168903220_275000_CN_315434352_275000/LConn1
  T_168903220_275000_/LConn2 -- _CN_168903220_275000_CN_315434352_275000/LConn2
  T_168903220_275000_/LConn3 -- _CN_168903220_275000_CN_315434352_275000/LConn3
  _CN_168903220_275000_CN_315434352_275000/RConn1 -- T_315434352__/LConn1 -- 中東京幹線_CN_315434352_275000_CN_152991099_275000/LConn1
  _CN_168903220_275000_CN_315434352_275000/RConn2 -- T_315434352__/LConn2 -- 中東京幹線_CN_315434352_275000_CN_152991099_275000/LConn2
  _CN_168903220_275000_CN_315434352_275000/RConn3 -- T_315434352__/LConn3 -- 中東京幹線_CN_315434352_275000_CN_152991099_275000/LConn3
  _CN_169031998_500000_CN_109850439_500000/RConn1 -- T_109850439_500000_/LConn1 -- 阿南紀北直流幹線_CN_109850439_500000_CN_217885658_500000/LConn1
  _CN_169031998_500000_CN_109850439_500000/RConn2 -- T_109850439_500000_/LConn2 -- 阿南紀北直流幹線_CN_109850439_500000_CN_217885658_500000/LConn2
  _CN_169031998_500000_CN_109850439_500000/RConn3 -- T_109850439_500000_/LConn3 -- 阿南紀北直流幹線_CN_109850439_500000_CN_217885658_500000/LConn3
  T_190734269_275000_/LConn1 -- _CN_161946848_275000_CN_190734269_275000/RConn1
  T_190734269_275000_/LConn2 -- _CN_161946848_275000_CN_190734269_275000/RConn2
  T_190734269_275000_/LConn3 -- _CN_161946848_275000_CN_190734269_275000/RConn3
  新古河線_(Shin_Koga_Sen)_CN_133135172_500000_CN_133641619_500000/RConn1 -- T_133135172_500000_新古河変電所/LConn1 -- 福島幹線_CN_133135172_500000_CN_168839127_500000/RConn1 -- 新京葉線_CN_133135172_500000_CN_168727982_500000/RConn1 -- 新京葉線_CN_133135172_500000_CN_151706977_500000/LConn1 -- 新筑波線_(Shin_Tsukuba_Sen)_CN_133135172_500000_CN_132913106_500000/LConn1
  新古河線_(Shin_Koga_Sen)_CN_133135172_500000_CN_133641619_500000/RConn2 -- T_133135172_500000_新古河変電所/LConn2 -- 福島幹線_CN_133135172_500000_CN_168839127_500000/RConn2 -- 新京葉線_CN_133135172_500000_CN_168727982_500000/RConn2 -- 新京葉線_CN_133135172_500000_CN_151706977_500000/LConn2 -- 新筑波線_(Shin_Tsukuba_Sen)_CN_133135172_500000_CN_132913106_500000/LConn2
  新古河線_(Shin_Koga_Sen)_CN_133135172_500000_CN_133641619_500000/RConn3 -- T_133135172_500000_新古河変電所/LConn3 -- 福島幹線_CN_133135172_500000_CN_168839127_500000/RConn3 -- 新京葉線_CN_133135172_500000_CN_168727982_500000/RConn3 -- 新京葉線_CN_133135172_500000_CN_151706977_500000/LConn3 -- 新筑波線_(Shin_Tsukuba_Sen)_CN_133135172_500000_CN_132913106_500000/LConn3
  T_151706977__新野田変電所_(Shin_Noda_Hendensho)/LConn1 -- 新京葉線_CN_133135172_500000_CN_151706977_500000/RConn1
  T_151706977__新野田変電所_(Shin_Noda_Hendensho)/LConn2 -- 新京葉線_CN_133135172_500000_CN_151706977_500000/RConn2
  T_151706977__新野田変電所_(Shin_Noda_Hendensho)/LConn3 -- 新京葉線_CN_133135172_500000_CN_151706977_500000/RConn3
  新筑波線_(Shin_Tsukuba_Sen)_CN_133135172_500000_CN_132913106_500000/RConn1 -- T_132913106_500000_新筑波変電所_(Shin_Tsukuba_Hendensho)/LConn1 -- 新佐原線_CN_132913106_500000_CN_105298089_500000/RConn1 -- _CN_132913106_500000_CN_104391636_500000/RConn1
  新筑波線_(Shin_Tsukuba_Sen)_CN_133135172_500000_CN_132913106_500000/RConn2 -- T_132913106_500000_新筑波変電所_(Shin_Tsukuba_Hendensho)/LConn2 -- 新佐原線_CN_132913106_500000_CN_105298089_500000/RConn2 -- _CN_132913106_500000_CN_104391636_500000/RConn2
  新筑波線_(Shin_Tsukuba_Sen)_CN_133135172_500000_CN_132913106_500000/RConn3 -- T_132913106_500000_新筑波変電所_(Shin_Tsukuba_Hendensho)/LConn3 -- 新佐原線_CN_132913106_500000_CN_105298089_500000/RConn3 -- _CN_132913106_500000_CN_104391636_500000/RConn3
  T_110682955_275000;154000;77000_伊丹変電所_(Itami_Hendensho)/LConn1 -- _CN_110682951_275000_CN_110682955_275000/RConn1
  T_110682955_275000;154000;77000_伊丹変電所_(Itami_Hendensho)/LConn2 -- _CN_110682951_275000_CN_110682955_275000/RConn2
  T_110682955_275000;154000;77000_伊丹変電所_(Itami_Hendensho)/LConn3 -- _CN_110682951_275000_CN_110682955_275000/RConn3
  T_185029969_500000;220000_/LConn1 -- _CN_185029969_500000_CN216798219/LConn1
  T_185029969_500000;220000_/LConn2 -- _CN_185029969_500000_CN216798219/LConn2
  T_185029969_500000;220000_/LConn3 -- _CN_185029969_500000_CN216798219/LConn3
  G_216798219_九州電力_松浦火力発電所/RConn1 -- _CN_185029969_500000_CN216798219/RConn1
  G_216798219_九州電力_松浦火力発電所/RConn2 -- _CN_185029969_500000_CN216798219/RConn2
  G_216798219_九州電力_松浦火力発電所/RConn3 -- _CN_185029969_500000_CN216798219/RConn3
  _CN_170605907_500000_CN_110682956_500000/RConn1 -- T_170605907_500000_北摂変電所/LConn1 -- _CN_170605907_500000_CN_241822631_500000/LConn1
  _CN_170605907_500000_CN_110682956_500000/RConn2 -- T_170605907_500000_北摂変電所/LConn2 -- _CN_170605907_500000_CN_241822631_500000/LConn2
  _CN_170605907_500000_CN_110682956_500000/RConn3 -- T_170605907_500000_北摂変電所/LConn3 -- _CN_170605907_500000_CN_241822631_500000/LConn3
  _CN_170605907_500000_CN_241822631_500000/RConn1 -- T_241822631__/LConn1 -- _CN_241822623_500000_CN_241822631_500000/RConn1 -- _CN_241822621_500000_CN_241822631_500000/RConn1
  _CN_170605907_500000_CN_241822631_500000/RConn2 -- T_241822631__/LConn2 -- _CN_241822623_500000_CN_241822631_500000/RConn2 -- _CN_241822621_500000_CN_241822631_500000/RConn2
  _CN_170605907_500000_CN_241822631_500000/RConn3 -- T_241822631__/LConn3 -- _CN_241822623_500000_CN_241822631_500000/RConn3 -- _CN_241822621_500000_CN_241822631_500000/RConn3
  T_316459359_275000_/LConn1 -- _CN_316459359_275000_CN_107262429_275000/RConn1
  T_316459359_275000_/LConn2 -- _CN_316459359_275000_CN_107262429_275000/RConn2
  T_316459359_275000_/LConn3 -- _CN_316459359_275000_CN_107262429_275000/RConn3
  T_144077272__/LConn1 -- _CN_151706977_275000_CN_144077272_275000/RConn1
  T_144077272__/LConn2 -- _CN_151706977_275000_CN_144077272_275000/RConn2
  T_144077272__/LConn3 -- _CN_151706977_275000_CN_144077272_275000/RConn3
  G_103783431_福島第一_原子力発電所/RConn1 -- _CN_106309481_500000_CN103783431/RConn1
  G_103783431_福島第一_原子力発電所/RConn2 -- _CN_106309481_500000_CN103783431/RConn2
  G_103783431_福島第一_原子力発電所/RConn3 -- _CN_106309481_500000_CN103783431/RConn3
  T_152991099__中東京変電所/LConn1 -- 中東京幹線_CN_315434352_275000_CN_152991099_275000/RConn1
  T_152991099__中東京変電所/LConn2 -- 中東京幹線_CN_315434352_275000_CN_152991099_275000/RConn2
  T_152991099__中東京変電所/LConn3 -- 中東京幹線_CN_315434352_275000_CN_152991099_275000/RConn3
  T_190984572_275000_/LConn1 -- _CN_190984572_275000_CN191382966/LConn1
  T_190984572_275000_/LConn2 -- _CN_190984572_275000_CN191382966/LConn2
  T_190984572_275000_/LConn3 -- _CN_190984572_275000_CN191382966/LConn3
  G_191382966_喜撰山水力発電所/RConn1 -- _CN_190984572_275000_CN191382966/RConn1
  G_191382966_喜撰山水力発電所/RConn2 -- _CN_190984572_275000_CN191382966/RConn2
  G_191382966_喜撰山水力発電所/RConn3 -- _CN_190984572_275000_CN191382966/RConn3
  T_209726348_500000_信濃変電所/LConn1 -- 信濃幹線_CN_209726348_500000_CN_209429410_500000/LConn1
  T_209726348_500000_信濃変電所/LConn2 -- 信濃幹線_CN_209726348_500000_CN_209429410_500000/LConn2
  T_209726348_500000_信濃変電所/LConn3 -- 信濃幹線_CN_209726348_500000_CN_209429410_500000/LConn3
  信濃幹線_CN_209726348_500000_CN_209429410_500000/RConn1 -- T_209429410_500000_南信変電所/LConn1 -- 南信幹線_CN_209429410_500000_CN_142662111_500000/RConn1
  信濃幹線_CN_209726348_500000_CN_209429410_500000/RConn2 -- T_209429410_500000_南信変電所/LConn2 -- 南信幹線_CN_209429410_500000_CN_142662111_500000/RConn2
  信濃幹線_CN_209726348_500000_CN_209429410_500000/RConn3 -- T_209429410_500000_南信変電所/LConn3 -- 南信幹線_CN_209429410_500000_CN_142662111_500000/RConn3
  T_315662839_500000_新信濃変電所/LConn1 -- _CN_195615141_500000_CN_315662839_500000/RConn1
  T_315662839_500000_新信濃変電所/LConn2 -- _CN_195615141_500000_CN_315662839_500000/RConn2
  T_315662839_500000_新信濃変電所/LConn3 -- _CN_195615141_500000_CN_315662839_500000/RConn3
  G_242706111_/RConn1 -- _CN_241822631_275000_CN242706111/RConn1
  G_242706111_/RConn2 -- _CN_241822631_275000_CN242706111/RConn2
  G_242706111_/RConn3 -- _CN_241822631_275000_CN242706111/RConn3
  T_217885658_500000;0_由良開閉所/LConn1 -- 阿南紀北直流幹線_CN_109850439_500000_CN_217885658_500000/RConn1
  T_217885658_500000;0_由良開閉所/LConn2 -- 阿南紀北直流幹線_CN_109850439_500000_CN_217885658_500000/RConn2
  T_217885658_500000;0_由良開閉所/LConn3 -- 阿南紀北直流幹線_CN_109850439_500000_CN_217885658_500000/RConn3
  T_318302348_275000_東上越変電所/LConn1 -- _CN_318302348_275000_CN319098734/RConn1
  T_318302348_275000_東上越変電所/LConn2 -- _CN_318302348_275000_CN319098734/RConn2
  T_318302348_275000_東上越変電所/LConn3 -- _CN_318302348_275000_CN319098734/RConn3
  G_233174201_/RConn1 -- _CN_232998815_275000_CN233174201/RConn1
  G_233174201_/RConn2 -- _CN_232998815_275000_CN233174201/RConn2
  G_233174201_/RConn3 -- _CN_232998815_275000_CN233174201/RConn3
  T_153760214__多摩変電所/LConn1 -- 只見幹線_CN_153760214_275000_CN_47110637_275000/RConn1
  T_153760214__多摩変電所/LConn2 -- 只見幹線_CN_153760214_275000_CN_47110637_275000/RConn2
  T_153760214__多摩変電所/LConn3 -- 只見幹線_CN_153760214_275000_CN_47110637_275000/RConn3
  T_315662816__/LConn1 -- _CN_315662816_275000_CN210658603/RConn1
  T_315662816__/LConn2 -- _CN_315662816_275000_CN210658603/RConn2
  T_315662816__/LConn3 -- _CN_315662816_275000_CN210658603/RConn3
  G_110340505_新神戸変電所/RConn1 -- _CN_185032690_275000_CN110340505/RConn1
  G_110340505_新神戸変電所/RConn2 -- _CN_185032690_275000_CN110340505/RConn2
  G_110340505_新神戸変電所/RConn3 -- _CN_185032690_275000_CN110340505/RConn3
  T_201293312_500000;220000_/RConn1 -- L_201293312/LConn1
  T_201293312_500000;220000_/RConn2 -- L_201293312/LConn2
  T_201293312_500000;220000_/RConn3 -- L_201293312/LConn3
  T_216778426_500000;220000_/RConn1 -- L_216778426/LConn1
  T_216778426_500000;220000_/RConn2 -- L_216778426/LConn2
  T_216778426_500000;220000_/RConn3 -- L_216778426/LConn3
  T_187988970_500000;220000_/RConn1 -- L_187988970/LConn1
  T_187988970_500000;220000_/RConn2 -- L_187988970/LConn2
  T_187988970_500000;220000_/RConn3 -- L_187988970/LConn3
  T_169121281__北豊田変電所_(Kita_Toyota_Hendensho)/RConn1 -- L_169121281/LConn1
  T_169121281__北豊田変電所_(Kita_Toyota_Hendensho)/RConn2 -- L_169121281/LConn2
  T_169121281__北豊田変電所_(Kita_Toyota_Hendensho)/RConn3 -- L_169121281/LConn3
  T_169121284_275000_/RConn1 -- L_169121284/LConn1
  T_169121284_275000_/RConn2 -- L_169121284/LConn2
  T_169121284_275000_/RConn3 -- L_169121284/LConn3
  T_104173570_500000_/RConn1 -- L_104173570/LConn1
  T_104173570_500000_/RConn2 -- L_104173570/LConn2
  T_104173570_500000_/RConn3 -- L_104173570/LConn3
  T_106309481_500000_新福島変電所/RConn1 -- L_106309481/LConn1
  T_106309481_500000_新福島変電所/RConn2 -- L_106309481/LConn2
  T_106309481_500000_新福島変電所/RConn3 -- L_106309481/LConn3
  T_116828675_275000_北相模変電所_(Kita_Sagami_Hendensho)/RConn1 -- L_116828675/LConn1
  T_116828675_275000_北相模変電所_(Kita_Sagami_Hendensho)/RConn2 -- L_116828675/LConn2
  T_116828675_275000_北相模変電所_(Kita_Sagami_Hendensho)/RConn3 -- L_116828675/LConn3
  T_169121278_275000_電源名古屋/RConn1 -- L_169121278/LConn1
  T_169121278_275000_電源名古屋/RConn2 -- L_169121278/LConn2
  T_169121278_275000_電源名古屋/RConn3 -- L_169121278/LConn3
  T_170503689__/RConn1 -- L_170503689/LConn1
  T_170503689__/RConn2 -- L_170503689/LConn2
  T_170503689__/RConn3 -- L_170503689/LConn3
  T_170436908__/RConn1 -- L_170436908/LConn1
  T_170436908__/RConn2 -- L_170436908/LConn2
  T_170436908__/RConn3 -- L_170436908/LConn3
  T_168857610__/RConn1 -- L_168857610/LConn1
  T_168857610__/RConn2 -- L_168857610/LConn2
  T_168857610__/RConn3 -- L_168857610/LConn3
  T_104530060__新栃木変電所/RConn1 -- L_104530060/LConn1
  T_104530060__新栃木変電所/RConn2 -- L_104530060/LConn2
  T_104530060__新栃木変電所/RConn3 -- L_104530060/LConn3
  T_193544791_500000_新西広島変電所_(Shin_Nishi_Hiroshima_Hendensho)/RConn1 -- L_193544791/LConn1
  T_193544791_500000_新西広島変電所_(Shin_Nishi_Hiroshima_Hendensho)/RConn2 -- L_193544791/LConn2
  T_193544791_500000_新西広島変電所_(Shin_Nishi_Hiroshima_Hendensho)/RConn3 -- L_193544791/LConn3
  T_170974371_500000_新広島変電所_(Shin_Hiroshima_Hendensho)/RConn1 -- L_170974371/LConn1
  T_170974371_500000_新広島変電所_(Shin_Hiroshima_Hendensho)/RConn2 -- L_170974371/LConn2
  T_170974371_500000_新広島変電所_(Shin_Hiroshima_Hendensho)/RConn3 -- L_170974371/LConn3
  T_242253500_500000_東山口変電所_(Higashi_Yamaguchi_Hendensho)/RConn1 -- L_242253500/LConn1
  T_242253500_500000_東山口変電所_(Higashi_Yamaguchi_Hendensho)/RConn2 -- L_242253500/LConn2
  T_242253500_500000_東山口変電所_(Higashi_Yamaguchi_Hendensho)/RConn3 -- L_242253500/LConn3
  T_317416612_500000_西島根変電所/RConn1 -- L_317416612/LConn1
  T_317416612_500000_西島根変電所/RConn2 -- L_317416612/LConn2
  T_317416612_500000_西島根変電所/RConn3 -- L_317416612/LConn3
  T_161727149_500000_新生駒変電所_(Shin_Ikoma_Hendensho)/RConn1 -- L_161727149/LConn1
  T_161727149_500000_新生駒変電所_(Shin_Ikoma_Hendensho)/RConn2 -- L_161727149/LConn2
  T_161727149_500000_新生駒変電所_(Shin_Ikoma_Hendensho)/RConn3 -- L_161727149/LConn3
  T_169031921_500000_西京都変電所_(Nishi_Kyōto_Hendensho)/RConn1 -- L_169031921/LConn1
  T_169031921_500000_西京都変電所_(Nishi_Kyōto_Hendensho)/RConn2 -- L_169031921/LConn2
  T_169031921_500000_西京都変電所_(Nishi_Kyōto_Hendensho)/RConn3 -- L_169031921/LConn3
  T_169359724_500000_信貴変電所_(Shingi_Hendensho)/RConn1 -- L_169359724/LConn1
  T_169359724_500000_信貴変電所_(Shingi_Hendensho)/RConn2 -- L_169359724/LConn2
  T_169359724_500000_信貴変電所_(Shingi_Hendensho)/RConn3 -- L_169359724/LConn3
  T_161870227_500000_南京都変電所_(Minami_Kyōto_Hendensho)/RConn1 -- L_161870227/LConn1
  T_161870227_500000_南京都変電所_(Minami_Kyōto_Hendensho)/RConn2 -- L_161870227/LConn2
  T_161870227_500000_南京都変電所_(Minami_Kyōto_Hendensho)/RConn3 -- L_161870227/LConn3
  T_216502300__九州電力_中九州変電所/RConn1 -- L_216502300/LConn1
  T_216502300__九州電力_中九州変電所/RConn2 -- L_216502300/LConn2
  T_216502300__九州電力_中九州変電所/RConn3 -- L_216502300/LConn3
  T_215451416_500000;220000_九州電力南九州変電所/RConn1 -- L_215451416/LConn1
  T_215451416_500000;220000_九州電力南九州変電所/RConn2 -- L_215451416/LConn2
  T_215451416_500000;220000_九州電力南九州変電所/RConn3 -- L_215451416/LConn3
  T_149843487_500000_新秦野変電所_(Shin_Hatano_Hendensho)/RConn1 -- L_149843487/LConn1
  T_149843487_500000_新秦野変電所_(Shin_Hatano_Hendensho)/RConn2 -- L_149843487/LConn2
  T_149843487_500000_新秦野変電所_(Shin_Hatano_Hendensho)/RConn3 -- L_149843487/LConn3
  T_150065045_500000_新富士変電所/RConn1 -- L_150065045/LConn1
  T_150065045_500000_新富士変電所/RConn2 -- L_150065045/LConn2
  T_150065045_500000_新富士変電所/RConn3 -- L_150065045/LConn3
  T_145079972_500000_新多摩変電所_(Shin_Tama_Substation)/RConn1 -- L_145079972/LConn1
  T_145079972_500000_新多摩変電所_(Shin_Tama_Substation)/RConn2 -- L_145079972/LConn2
  T_145079972_500000_新多摩変電所_(Shin_Tama_Substation)/RConn3 -- L_145079972/LConn3
  T_162844704_275000_中相模変電所/RConn1 -- L_162844704/LConn1
  T_162844704_275000_中相模変電所/RConn2 -- L_162844704/LConn2
  T_162844704_275000_中相模変電所/RConn3 -- L_162844704/LConn3
  T_128364781_275000_東京電力_京浜変電所/RConn1 -- L_128364781/LConn1
  T_128364781_275000_東京電力_京浜変電所/RConn2 -- L_128364781/LConn2
  T_128364781_275000_東京電力_京浜変電所/RConn3 -- L_128364781/LConn3
  T_150035494_500000_/RConn1 -- L_150035494/LConn1
  T_150035494_500000_/RConn2 -- L_150035494/LConn2
  T_150035494_500000_/RConn3 -- L_150035494/LConn3
  T_66098469_500000_西群馬開閉所/RConn1 -- L_66098469/LConn1
  T_66098469_500000_西群馬開閉所/RConn2 -- L_66098469/LConn2
  T_66098469_500000_西群馬開閉所/RConn3 -- L_66098469/LConn3
  T_341208725__/RConn1 -- L_341208725/LConn1
  T_341208725__/RConn2 -- L_341208725/LConn2
  T_341208725__/RConn3 -- L_341208725/LConn3
  T_340647463__/RConn1 -- L_340647463/LConn1
  T_340647463__/RConn2 -- L_340647463/LConn2
  T_340647463__/RConn3 -- L_340647463/LConn3
  T_340648895__/RConn1 -- L_340648895/LConn1
  T_340648895__/RConn2 -- L_340648895/LConn2
  T_340648895__/RConn3 -- L_340648895/LConn3
  T_168852840__/RConn1 -- L_168852840/LConn1
  T_168852840__/RConn2 -- L_168852840/LConn2
  T_168852840__/RConn3 -- L_168852840/LConn3
  T_340647468__/RConn1 -- L_340647468/LConn1
  T_340647468__/RConn2 -- L_340647468/LConn2
  T_340647468__/RConn3 -- L_340647468/LConn3
  T_170589736_500000_東近江/RConn1 -- L_170589736/LConn1
  T_170589736_500000_東近江/RConn2 -- L_170589736/LConn2
  T_170589736_500000_東近江/RConn3 -- L_170589736/LConn3
  T_170568495_500000_三重開閉所/RConn1 -- L_170568495/LConn1
  T_170568495_500000_三重開閉所/RConn2 -- L_170568495/LConn2
  T_170568495_500000_三重開閉所/RConn3 -- L_170568495/LConn3
  T_319300956_275000_中越変電所/RConn1 -- L_319300956/LConn1
  T_319300956_275000_中越変電所/RConn2 -- L_319300956/LConn2
  T_319300956_275000_中越変電所/RConn3 -- L_319300956/LConn3
  T_318218831_275000_/RConn1 -- L_318218831/LConn1
  T_318218831_275000_/RConn2 -- L_318218831/LConn2
  T_318218831_275000_/RConn3 -- L_318218831/LConn3
  T_170537514_500000_/RConn1 -- L_170537514/LConn1
  T_170537514_500000_/RConn2 -- L_170537514/LConn2
  T_170537514_500000_/RConn3 -- L_170537514/LConn3
  T_192745005_275000_丸山変電所_(Maruyama_Hendensho)/RConn1 -- L_192745005/LConn1
  T_192745005_275000_丸山変電所_(Maruyama_Hendensho)/RConn2 -- L_192745005/LConn2
  T_192745005_275000_丸山変電所_(Maruyama_Hendensho)/RConn3 -- L_192745005/LConn3
  T_161946848_275000_関開閉所_(Seki)/RConn1 -- L_161946848/LConn1
  T_161946848_275000_関開閉所_(Seki)/RConn2 -- L_161946848/LConn2
  T_161946848_275000_関開閉所_(Seki)/RConn3 -- L_161946848/LConn3
  T_108199478_275000_南大阪変電所_(Minamiōsaka_Hendensho)/RConn1 -- L_108199478/LConn1
  T_108199478_275000_南大阪変電所_(Minamiōsaka_Hendensho)/RConn2 -- L_108199478/LConn2
  T_108199478_275000_南大阪変電所_(Minamiōsaka_Hendensho)/RConn3 -- L_108199478/LConn3
  T_109834508_275000_金剛開閉所_(Kongō_Kaiheisho)/RConn1 -- L_109834508/LConn1
  T_109834508_275000_金剛開閉所_(Kongō_Kaiheisho)/RConn2 -- L_109834508/LConn2
  T_109834508_275000_金剛開閉所_(Kongō_Kaiheisho)/RConn3 -- L_109834508/LConn3
  T_158522649_275000_東大阪変電所/RConn1 -- L_158522649/LConn1
  T_158522649_275000_東大阪変電所/RConn2 -- L_158522649/LConn2
  T_158522649_275000_東大阪変電所/RConn3 -- L_158522649/LConn3
  T_315614776_275000_/RConn1 -- L_315614776/LConn1
  T_315614776_275000_/RConn2 -- L_315614776/LConn2
  T_315614776_275000_/RConn3 -- L_315614776/LConn3
  T_315614783_275000_/RConn1 -- L_315614783/LConn1
  T_315614783_275000_/RConn2 -- L_315614783/LConn2
  T_315614783_275000_/RConn3 -- L_315614783/LConn3
  T_316566585_275000_/RConn1 -- L_316566585/LConn1
  T_316566585_275000_/RConn2 -- L_316566585/LConn2
  T_316566585_275000_/RConn3 -- L_316566585/LConn3
  T_174636874_275000_岩手変電所/RConn1 -- L_174636874/LConn1
  T_174636874_275000_岩手変電所/RConn2 -- L_174636874/LConn2
  T_174636874_275000_岩手変電所/RConn3 -- L_174636874/LConn3
  T_316566588_275000_/RConn1 -- L_316566588/LConn1
  T_316566588_275000_/RConn2 -- L_316566588/LConn2
  T_316566588_275000_/RConn3 -- L_316566588/LConn3
  T_316581632_275000_/RConn1 -- L_316581632/LConn1
  T_316581632_275000_/RConn2 -- L_316581632/LConn2
  T_316581632_275000_/RConn3 -- L_316581632/LConn3
  T_308348224_275000_新庄変電所/RConn1 -- L_308348224/LConn1
  T_308348224_275000_新庄変電所/RConn2 -- L_308348224/LConn2
  T_308348224_275000_新庄変電所/RConn3 -- L_308348224/LConn3
  T_256682313__/RConn1 -- L_256682313/LConn1
  T_256682313__/RConn2 -- L_256682313/LConn2
  T_256682313__/RConn3 -- L_256682313/LConn3
  T_116559939_500000_/RConn1 -- L_116559939/LConn1
  T_116559939_500000_/RConn2 -- L_116559939/LConn2
  T_116559939_500000_/RConn3 -- L_116559939/LConn3
  T_210090094_500000_駿遠変電所/RConn1 -- L_210090094/LConn1
  T_210090094_500000_駿遠変電所/RConn2 -- L_210090094/LConn2
  T_210090094_500000_駿遠変電所/RConn3 -- L_210090094/LConn3
  T_103818820_275000_仙台変電所/RConn1 -- L_103818820/LConn1
  T_103818820_275000_仙台変電所/RConn2 -- L_103818820/LConn2
  T_103818820_275000_仙台変電所/RConn3 -- L_103818820/LConn3
  T_250430935_275000_米沢変電所_(Yonezawa_Hendensho)/RConn1 -- L_250430935/LConn1
  T_250430935_275000_米沢変電所_(Yonezawa_Hendensho)/RConn2 -- L_250430935/LConn2
  T_250430935_275000_米沢変電所_(Yonezawa_Hendensho)/RConn3 -- L_250430935/LConn3
  T_172601929_500000;220000_/RConn1 -- L_172601929/LConn1
  T_172601929_500000;220000_/RConn2 -- L_172601929/LConn2
  T_172601929_500000;220000_/RConn3 -- L_172601929/LConn3
  T_186510275_500000_3_4号_開閉所/RConn1 -- L_186510275/LConn1
  T_186510275_500000_3_4号_開閉所/RConn2 -- L_186510275/LConn2
  T_186510275_500000_3_4号_開閉所/RConn3 -- L_186510275/LConn3
  T_327974991__東京電力逗子変電所/RConn1 -- L_327974991/LConn1
  T_327974991__東京電力逗子変電所/RConn2 -- L_327974991/LConn2
  T_327974991__東京電力逗子変電所/RConn3 -- L_327974991/LConn3
  T_158064651_275000_田子倉発電所/RConn1 -- L_158064651/LConn1
  T_158064651_275000_田子倉発電所/RConn2 -- L_158064651/LConn2
  T_158064651_275000_田子倉発電所/RConn3 -- L_158064651/LConn3
  T_232998815_275000_/RConn1 -- L_232998815/LConn1
  T_232998815_275000_/RConn2 -- L_232998815/LConn2
  T_232998815_275000_/RConn3 -- L_232998815/LConn3
  T_169122898_500000_東部変電所/RConn1 -- L_169122898/LConn1
  T_169122898_500000_東部変電所/RConn2 -- L_169122898/LConn2
  T_169122898_500000_東部変電所/RConn3 -- L_169122898/LConn3
  T_170247312_500000_新三河/RConn1 -- L_170247312/LConn1
  T_170247312_500000_新三河/RConn2 -- L_170247312/LConn2
  T_170247312_500000_新三河/RConn3 -- L_170247312/LConn3
  T_142662111_500000_中部電力㈱豊根開閉所/RConn1 -- L_142662111/LConn1
  T_142662111_500000_中部電力㈱豊根開閉所/RConn2 -- L_142662111/LConn2
  T_142662111_500000_中部電力㈱豊根開閉所/RConn3 -- L_142662111/LConn3
  T_170366035_500000_/RConn1 -- L_170366035/LConn1
  T_170366035_500000_/RConn2 -- L_170366035/LConn2
  T_170366035_500000_/RConn3 -- L_170366035/LConn3
  T_170850727_500000_愛知変電所/RConn1 -- L_170850727/LConn1
  T_170850727_500000_愛知変電所/RConn2 -- L_170850727/LConn2
  T_170850727_500000_愛知変電所/RConn3 -- L_170850727/LConn3
  T_170366036_275000_東豊田変電所/RConn1 -- L_170366036/LConn1
  T_170366036_275000_東豊田変電所/RConn2 -- L_170366036/LConn2
  T_170366036_275000_東豊田変電所/RConn3 -- L_170366036/LConn3
  T_170247359_275000_/RConn1 -- L_170247359/LConn1
  T_170247359_275000_/RConn2 -- L_170247359/LConn2
  T_170247359_275000_/RConn3 -- L_170247359/LConn3
  T_170366038_275000_/RConn1 -- L_170366038/LConn1
  T_170366038_275000_/RConn2 -- L_170366038/LConn2
  T_170366038_275000_/RConn3 -- L_170366038/LConn3
  T_241956440_275000_伊勢開閉所/RConn1 -- L_241956440/LConn1
  T_241956440_275000_伊勢開閉所/RConn2 -- L_241956440/LConn2
  T_241956440_275000_伊勢開閉所/RConn3 -- L_241956440/LConn3
  T_242532736_275000_/RConn1 -- L_242532736/LConn1
  T_242532736_275000_/RConn2 -- L_242532736/LConn2
  T_242532736_275000_/RConn3 -- L_242532736/LConn3
  T_170793703_275000_西尾張/RConn1 -- L_170793703/LConn1
  T_170793703_275000_西尾張/RConn2 -- L_170793703/LConn2
  T_170793703_275000_西尾張/RConn3 -- L_170793703/LConn3
  T_241923317_275000_南勢変電所_(Nansei_Hendensho)/RConn1 -- L_241923317/LConn1
  T_241923317_275000_南勢変電所_(Nansei_Hendensho)/RConn2 -- L_241923317/LConn2
  T_241923317_275000_南勢変電所_(Nansei_Hendensho)/RConn3 -- L_241923317/LConn3
  T_169993955_275000_新潟変電所/RConn1 -- L_169993955/LConn1
  T_169993955_275000_新潟変電所/RConn2 -- L_169993955/LConn2
  T_169993955_275000_新潟変電所/RConn3 -- L_169993955/LConn3
  T_170016148_275000_北新潟変電所/RConn1 -- L_170016148/LConn1
  T_170016148_275000_北新潟変電所/RConn2 -- L_170016148/LConn2
  T_170016148_275000_北新潟変電所/RConn3 -- L_170016148/LConn3
  T_133137636_275000_北東京変電所_(Kita_Tōkyō_Hendensho)/RConn1 -- L_133137636/LConn1
  T_133137636_275000_北東京変電所_(Kita_Tōkyō_Hendensho)/RConn2 -- L_133137636/LConn2
  T_133137636_275000_北東京変電所_(Kita_Tōkyō_Hendensho)/RConn3 -- L_133137636/LConn3
  T_128581912_500000;275000;66000_新坂戸変電所/RConn4 -- L_128581912/LConn1
  T_128581912_500000;275000;66000_新坂戸変電所/RConn5 -- L_128581912/LConn2
  T_128581912_500000;275000;66000_新坂戸変電所/RConn6 -- L_128581912/LConn3
  T_151706977__新野田変電所_(Shin_Noda_Hendensho)/RConn4 -- L_151706977/LConn1
  T_151706977__新野田変電所_(Shin_Noda_Hendensho)/RConn5 -- L_151706977/LConn2
  T_151706977__新野田変電所_(Shin_Noda_Hendensho)/RConn6 -- L_151706977/LConn3
  T_155411568__/RConn1 -- L_155411568/LConn1
  T_155411568__/RConn2 -- L_155411568/LConn2
  T_155411568__/RConn3 -- L_155411568/LConn3
  T_145084773_275000_青梅変電所/RConn1 -- L_145084773/LConn1
  T_145084773_275000_青梅変電所/RConn2 -- L_145084773/LConn2
  T_145084773_275000_青梅変電所/RConn3 -- L_145084773/LConn3
  T_133644487__/RConn1 -- L_133644487/LConn1
  T_133644487__/RConn2 -- L_133644487/LConn2
  T_133644487__/RConn3 -- L_133644487/LConn3
  T_262597734__海部開閉所/RConn1 -- L_262597734/LConn1
  T_262597734__海部開閉所/RConn2 -- L_262597734/LConn2
  T_262597734__海部開閉所/RConn3 -- L_262597734/LConn3
  T_87682157_275000_南川越変電所_(Minamikawagoe_Hendensho)/RConn1 -- L_87682157/LConn1
  T_87682157_275000_南川越変電所_(Minamikawagoe_Hendensho)/RConn2 -- L_87682157/LConn2
  T_87682157_275000_南川越変電所_(Minamikawagoe_Hendensho)/RConn3 -- L_87682157/LConn3
  T_159491797_275000_南狭山変電所_(Minamisayama_Hendensho)/RConn1 -- L_159491797/LConn1
  T_159491797_275000_南狭山変電所_(Minamisayama_Hendensho)/RConn2 -- L_159491797/LConn2
  T_159491797_275000_南狭山変電所_(Minamisayama_Hendensho)/RConn3 -- L_159491797/LConn3
  T_105291887_275000_那珂変電所_(Naka_Hendensho)/RConn1 -- L_105291887/LConn1
  T_105291887_275000_那珂変電所_(Naka_Hendensho)/RConn2 -- L_105291887/LConn2
  T_105291887_275000_那珂変電所_(Naka_Hendensho)/RConn3 -- L_105291887/LConn3
  T_168839127__新茂木/RConn4 -- L_168839127/LConn1
  T_168839127__新茂木/RConn5 -- L_168839127/LConn2
  T_168839127__新茂木/RConn6 -- L_168839127/LConn3
  T_153521822_275000_西越谷変電所_(Nishi_Koshigaya_Hendensho)/RConn1 -- L_153521822/LConn1
  T_153521822_275000_西越谷変電所_(Nishi_Koshigaya_Hendensho)/RConn2 -- L_153521822/LConn2
  T_153521822_275000_西越谷変電所_(Nishi_Koshigaya_Hendensho)/RConn3 -- L_153521822/LConn3
  T_315434358_500000_新岡部変電所/RConn1 -- L_315434358/LConn1
  T_315434358_500000_新岡部変電所/RConn2 -- L_315434358/LConn2
  T_315434358_500000_新岡部変電所/RConn3 -- L_315434358/LConn3
  T_320438391_500000_/RConn1 -- L_320438391/LConn1
  T_320438391_500000_/RConn2 -- L_320438391/LConn2
  T_320438391_500000_/RConn3 -- L_320438391/LConn3
  T_241822621_500000_/RConn1 -- L_241822621/LConn1
  T_241822621_500000_/RConn2 -- L_241822621/LConn2
  T_241822621_500000_/RConn3 -- L_241822621/LConn3
  T_110682956_500000_猪名川変電所/RConn1 -- L_110682956/LConn1
  T_110682956_500000_猪名川変電所/RConn2 -- L_110682956/LConn2
  T_110682956_500000_猪名川変電所/RConn3 -- L_110682956/LConn3
  T_320444665_500000_/RConn1 -- L_320444665/LConn1
  T_320444665_500000_/RConn2 -- L_320444665/LConn2
  T_320444665_500000_/RConn3 -- L_320444665/LConn3
  T_179417733_275000_/RConn1 -- L_179417733/LConn1
  T_179417733_275000_/RConn2 -- L_179417733/LConn2
  T_179417733_275000_/RConn3 -- L_179417733/LConn3
  T_161948515_275000_西濃変電所_(Seinō_Hendensho)/RConn1 -- L_161948515/LConn1
  T_161948515_275000_西濃変電所_(Seinō_Hendensho)/RConn2 -- L_161948515/LConn2
  T_161948515_275000_西濃変電所_(Seinō_Hendensho)/RConn3 -- L_161948515/LConn3
  T_315461259_500000_/RConn1 -- L_315461259/LConn1
  T_315461259_500000_/RConn2 -- L_315461259/LConn2
  T_315461259_500000_/RConn3 -- L_315461259/LConn3
  T_315461272_500000_新木更津変電所/RConn1 -- L_315461272/LConn1
  T_315461272_500000_新木更津変電所/RConn2 -- L_315461272/LConn2
  T_315461272_500000_新木更津変電所/RConn3 -- L_315461272/LConn3
  T_170247308_275000_三河変電所/RConn1 -- L_170247308/LConn1
  T_170247308_275000_三河変電所/RConn2 -- L_170247308/LConn2
  T_170247308_275000_三河変電所/RConn3 -- L_170247308/LConn3
  T_170260165_275000_中部電力湖西変電所/RConn1 -- L_170260165/LConn1
  T_170260165_275000_中部電力湖西変電所/RConn2 -- L_170260165/LConn2
  T_170260165_275000_中部電力湖西変電所/RConn3 -- L_170260165/LConn3
  T_133641619_500000_新所沢変電所_(Shin_Tokorozawa_Hendensho)/RConn1 -- L_133641619/LConn1
  T_133641619_500000_新所沢変電所_(Shin_Tokorozawa_Hendensho)/RConn2 -- L_133641619/LConn2
  T_133641619_500000_新所沢変電所_(Shin_Tokorozawa_Hendensho)/RConn3 -- L_133641619/LConn3
  T_170247314_275000_額田開閉所/RConn1 -- L_170247314/LConn1
  T_170247314_275000_額田開閉所/RConn2 -- L_170247314/LConn2
  T_170247314_275000_額田開閉所/RConn3 -- L_170247314/LConn3
  T_315608215_500000_/RConn1 -- L_315608215/LConn1
  T_315608215_500000_/RConn2 -- L_315608215/LConn2
  T_315608215_500000_/RConn3 -- L_315608215/LConn3
  T_169249243_500000_南福光変電所/RConn1 -- L_169249243/LConn1
  T_169249243_500000_南福光変電所/RConn2 -- L_169249243/LConn2
  T_169249243_500000_南福光変電所/RConn3 -- L_169249243/LConn3
  T_169249247_500000_加賀変電所/RConn1 -- L_169249247/LConn1
  T_169249247_500000_加賀変電所/RConn2 -- L_169249247/LConn2
  T_169249247_500000_加賀変電所/RConn3 -- L_169249247/LConn3
  T_105298089_500000_新佐原変電所/RConn1 -- L_105298089/LConn1
  T_105298089_500000_新佐原変電所/RConn2 -- L_105298089/LConn2
  T_105298089_500000_新佐原変電所/RConn3 -- L_105298089/LConn3
  T_302164677__秋田変電所/RConn1 -- L_302164677/LConn1
  T_302164677__秋田変電所/RConn2 -- L_302164677/LConn2
  T_302164677__秋田変電所/RConn3 -- L_302164677/LConn3
  T_316727625_275000_/RConn1 -- L_316727625/LConn1
  T_316727625_275000_/RConn2 -- L_316727625/LConn2
  T_316727625_275000_/RConn3 -- L_316727625/LConn3
  T_302164679_275000_能代変電所/RConn1 -- L_302164679/LConn1
  T_302164679_275000_能代変電所/RConn2 -- L_302164679/LConn2
  T_302164679_275000_能代変電所/RConn3 -- L_302164679/LConn3
  T_241828221_500000_新岡山変電所_(Shin_Okayama_Hendensho)/RConn1 -- L_241828221/LConn1
  T_241828221_500000_新岡山変電所_(Shin_Okayama_Hendensho)/RConn2 -- L_241828221/LConn2
  T_241828221_500000_新岡山変電所_(Shin_Okayama_Hendensho)/RConn3 -- L_241828221/LConn3
  T_242103481_500000_日野変電所/RConn1 -- L_242103481/LConn1
  T_242103481_500000_日野変電所/RConn2 -- L_242103481/LConn2
  T_242103481_500000_日野変電所/RConn3 -- L_242103481/LConn3
  T_204258596_500000_/RConn1 -- L_204258596/LConn1
  T_204258596_500000_/RConn2 -- L_204258596/LConn2
  T_204258596_500000_/RConn3 -- L_204258596/LConn3
  T_315757225_275000_/RConn1 -- L_315757225/LConn1
  T_315757225_275000_/RConn2 -- L_315757225/LConn2
  T_315757225_275000_/RConn3 -- L_315757225/LConn3
  T_316581637_275000_青森変電所/RConn1 -- L_316581637/LConn1
  T_316581637_275000_青森変電所/RConn2 -- L_316581637/LConn2
  T_316581637_275000_青森変電所/RConn3 -- L_316581637/LConn3
  T_87538349_500000_讃岐変電所/RConn1 -- L_87538349/LConn1
  T_87538349_500000_讃岐変電所/RConn2 -- L_87538349/LConn2
  T_87538349_500000_讃岐変電所/RConn3 -- L_87538349/LConn3
  T_171066843_500000_四国電力東予変電所/RConn1 -- L_171066843/LConn1
  T_171066843_500000_四国電力東予変電所/RConn2 -- L_171066843/LConn2
  T_171066843_500000_四国電力東予変電所/RConn3 -- L_171066843/LConn3
  T_102958903_500000_/RConn1 -- L_102958903/LConn1
  T_102958903_500000_/RConn2 -- L_102958903/LConn2
  T_102958903_500000_/RConn3 -- L_102958903/LConn3
  T_242253497_275000_姫路変電所_(Himeji_Hendensho)/RConn1 -- L_242253497/LConn1
  T_242253497_275000_姫路変電所_(Himeji_Hendensho)/RConn2 -- L_242253497/LConn2
  T_242253497_275000_姫路変電所_(Himeji_Hendensho)/RConn3 -- L_242253497/LConn3
  T_185032690_275000_西神戸変電所/RConn1 -- L_185032690/LConn1
  T_185032690_275000_西神戸変電所/RConn2 -- L_185032690/LConn2
  T_185032690_275000_西神戸変電所/RConn3 -- L_185032690/LConn3
  T_241822631__/RConn4 -- L_241822631/LConn1
  T_241822631__/RConn5 -- L_241822631/LConn2
  T_241822631__/RConn6 -- L_241822631/LConn3
  T_160374974_275000;77000_北葛城変電所_(Kita_Katsuragi_Hendensho)/RConn1 -- L_160374974/LConn1
  T_160374974_275000;77000_北葛城変電所_(Kita_Katsuragi_Hendensho)/RConn2 -- L_160374974/LConn2
  T_160374974_275000;77000_北葛城変電所_(Kita_Katsuragi_Hendensho)/RConn3 -- L_160374974/LConn3
  T_216956620_500000_/RConn1 -- L_216956620/LConn1
  T_216956620_500000_/RConn2 -- L_216956620/LConn2
  T_216956620_500000_/RConn3 -- L_216956620/LConn3
  T_159191758_275000_北松本変電所/RConn1 -- L_159191758/LConn1
  T_159191758_275000_北松本変電所/RConn2 -- L_159191758/LConn2
  T_159191758_275000_北松本変電所/RConn3 -- L_159191758/LConn3
  T_211258348_275000_東信変電所/RConn1 -- L_211258348/LConn1
  T_211258348_275000_東信変電所/RConn2 -- L_211258348/LConn2
  T_211258348_275000_東信変電所/RConn3 -- L_211258348/LConn3
  T_253566674__/RConn1 -- L_253566674/LConn1
  T_253566674__/RConn2 -- L_253566674/LConn2
  T_253566674__/RConn3 -- L_253566674/LConn3
  T_104391636_500000_新いわき/RConn1 -- L_104391636/LConn1
  T_104391636_500000_新いわき/RConn2 -- L_104391636/LConn2
  T_104391636_500000_新いわき/RConn3 -- L_104391636/LConn3
  T_156208858_500000_南相馬変電所/RConn1 -- L_156208858/LConn1
  T_156208858_500000_南相馬変電所/RConn2 -- L_156208858/LConn2
  T_156208858_500000_南相馬変電所/RConn3 -- L_156208858/LConn3
  T_136298957__新座変電所/RConn1 -- L_136298957/LConn1
  T_136298957__新座変電所/RConn2 -- L_136298957/LConn2
  T_136298957__新座変電所/RConn3 -- L_136298957/LConn3
  T_169963227_500000_新榛名/RConn1 -- L_169963227/LConn1
  T_169963227_500000_新榛名/RConn2 -- L_169963227/LConn2
  T_169963227_500000_新榛名/RConn3 -- L_169963227/LConn3
  T_169963236__/RConn1 -- L_169963236/LConn1
  T_169963236__/RConn2 -- L_169963236/LConn2
  T_169963236__/RConn3 -- L_169963236/LConn3
  T_195615141_500000_/RConn1 -- L_195615141/LConn1
  T_195615141_500000_/RConn2 -- L_195615141/LConn2
  T_195615141_500000_/RConn3 -- L_195615141/LConn3
  T_199544541_275000_新北信変電所/RConn1 -- L_199544541/LConn1
  T_199544541_275000_新北信変電所/RConn2 -- L_199544541/LConn2
  T_199544541_275000_新北信変電所/RConn3 -- L_199544541/LConn3
  T_317511904_500000_北松江変電所/RConn1 -- L_317511904/LConn1
  T_317511904_500000_北松江変電所/RConn2 -- L_317511904/LConn2
  T_317511904_500000_北松江変電所/RConn3 -- L_317511904/LConn3
  T_242253537__/RConn1 -- L_242253537/LConn1
  T_242253537__/RConn2 -- L_242253537/LConn2
  T_242253537__/RConn3 -- L_242253537/LConn3
  T_210765350__花見川変電所_(Hanamigawa_Hendensho)/RConn1 -- L_210765350/LConn1
  T_210765350__花見川変電所_(Hanamigawa_Hendensho)/RConn2 -- L_210765350/LConn2
  T_210765350__花見川変電所_(Hanamigawa_Hendensho)/RConn3 -- L_210765350/LConn3
  T_211241774__/RConn1 -- L_211241774/LConn1
  T_211241774__/RConn2 -- L_211241774/LConn2
  T_211241774__/RConn3 -- L_211241774/LConn3
  T_170793702_275000_西名古屋/RConn1 -- L_170793702/LConn1
  T_170793702_275000_西名古屋/RConn2 -- L_170793702/LConn2
  T_170793702_275000_西名古屋/RConn3 -- L_170793702/LConn3
  T_179863079_275000_/RConn1 -- L_179863079/LConn1
  T_179863079_275000_/RConn2 -- L_179863079/LConn2
  T_179863079_275000_/RConn3 -- L_179863079/LConn3
  T_256894928__/RConn1 -- L_256894928/LConn1
  T_256894928__/RConn2 -- L_256894928/LConn2
  T_256894928__/RConn3 -- L_256894928/LConn3
  T_168524732__/RConn1 -- L_168524732/LConn1
  T_168524732__/RConn2 -- L_168524732/LConn2
  T_168524732__/RConn3 -- L_168524732/LConn3
  T_242103532_500000_/RConn1 -- L_242103532/LConn1
  T_242103532_500000_/RConn2 -- L_242103532/LConn2
  T_242103532_500000_/RConn3 -- L_242103532/LConn3
  T_241822623_500000;220000;110000_/RConn1 -- L_241822623/LConn1
  T_241822623_500000;220000;110000_/RConn2 -- L_241822623/LConn2
  T_241822623_500000;220000;110000_/RConn3 -- L_241822623/LConn3
  T_47110637_275000_西東京変電所/RConn1 -- L_47110637/LConn1
  T_47110637_275000_西東京変電所/RConn2 -- L_47110637/LConn2
  T_47110637_275000_西東京変電所/RConn3 -- L_47110637/LConn3
  T_169031922__/RConn1 -- L_169031922/LConn1
  T_169031922__/RConn2 -- L_169031922/LConn2
  T_169031922__/RConn3 -- L_169031922/LConn3
  T_169031998__/RConn1 -- L_169031998/LConn1
  T_169031998__/RConn2 -- L_169031998/LConn2
  T_169031998__/RConn3 -- L_169031998/LConn3
  T_104375141_275000_須賀川変電所_(Sukagawa_Hendensho)/RConn1 -- L_104375141/LConn1
  T_104375141_275000_須賀川変電所_(Sukagawa_Hendensho)/RConn2 -- L_104375141/LConn2
  T_104375141_275000_須賀川変電所_(Sukagawa_Hendensho)/RConn3 -- L_104375141/LConn3
  T_107262429_275000_福島変電所/RConn1 -- L_107262429/LConn1
  T_107262429_275000_福島変電所/RConn2 -- L_107262429/LConn2
  T_107262429_275000_福島変電所/RConn3 -- L_107262429/LConn3
  T_250540807_500000_東群馬変電所_(Higashi_Gunma_Substation)/RConn1 -- L_250540807/LConn1
  T_250540807_500000_東群馬変電所_(Higashi_Gunma_Substation)/RConn2 -- L_250540807/LConn2
  T_250540807_500000_東群馬変電所_(Higashi_Gunma_Substation)/RConn3 -- L_250540807/LConn3
  T_291678103_275000_紀の川変電所_(Kinokawa_Hendensho)/RConn1 -- L_291678103/LConn1
  T_291678103_275000_紀の川変電所_(Kinokawa_Hendensho)/RConn2 -- L_291678103/LConn2
  T_291678103_275000_紀の川変電所_(Kinokawa_Hendensho)/RConn3 -- L_291678103/LConn3
  T_151379730_500000_房総変電所_(Bōsō_Hendensho)/RConn1 -- L_151379730/LConn1
  T_151379730_500000_房総変電所_(Bōsō_Hendensho)/RConn2 -- L_151379730/LConn2
  T_151379730_500000_房総変電所_(Bōsō_Hendensho)/RConn3 -- L_151379730/LConn3
  T_168727982_500000_新京葉変電所/RConn1 -- L_168727982/LConn1
  T_168727982_500000_新京葉変電所/RConn2 -- L_168727982/LConn2
  T_168727982_500000_新京葉変電所/RConn3 -- L_168727982/LConn3
  T_325868333_275000_/RConn1 -- L_325868333/LConn1
  T_325868333_275000_/RConn2 -- L_325868333/LConn2
  T_325868333_275000_/RConn3 -- L_325868333/LConn3
  T_110682951_275000_宝塚開閉所_(Takarazuka_Kaiheisho)/RConn1 -- L_110682951/LConn1
  T_110682951_275000_宝塚開閉所_(Takarazuka_Kaiheisho)/RConn2 -- L_110682951/LConn2
  T_110682951_275000_宝塚開閉所_(Takarazuka_Kaiheisho)/RConn3 -- L_110682951/LConn3
  T_145080115_275000_/RConn1 -- L_145080115/LConn1
  T_145080115_275000_/RConn2 -- L_145080115/LConn2
  T_145080115_275000_/RConn3 -- L_145080115/LConn3
  T_168903220_275000_/RConn1 -- L_168903220/LConn1
  T_168903220_275000_/RConn2 -- L_168903220/LConn2
  T_168903220_275000_/RConn3 -- L_168903220/LConn3
  T_315434352__/RConn1 -- L_315434352/LConn1
  T_315434352__/RConn2 -- L_315434352/LConn2
  T_315434352__/RConn3 -- L_315434352/LConn3
  T_109850439_500000_/RConn1 -- L_109850439/LConn1
  T_109850439_500000_/RConn2 -- L_109850439/LConn2
  T_109850439_500000_/RConn3 -- L_109850439/LConn3
  T_190734269_275000_/RConn1 -- L_190734269/LConn1
  T_190734269_275000_/RConn2 -- L_190734269/LConn2
  T_190734269_275000_/RConn3 -- L_190734269/LConn3
  T_133135172_500000_新古河変電所/RConn1 -- L_133135172/LConn1
  T_133135172_500000_新古河変電所/RConn2 -- L_133135172/LConn2
  T_133135172_500000_新古河変電所/RConn3 -- L_133135172/LConn3
  T_132913106_500000_新筑波変電所_(Shin_Tsukuba_Hendensho)/RConn1 -- L_132913106/LConn1
  T_132913106_500000_新筑波変電所_(Shin_Tsukuba_Hendensho)/RConn2 -- L_132913106/LConn2
  T_132913106_500000_新筑波変電所_(Shin_Tsukuba_Hendensho)/RConn3 -- L_132913106/LConn3
  T_110682955_275000;154000;77000_伊丹変電所_(Itami_Hendensho)/RConn1 -- L_110682955/LConn1
  T_110682955_275000;154000;77000_伊丹変電所_(Itami_Hendensho)/RConn2 -- L_110682955/LConn2
  T_110682955_275000;154000;77000_伊丹変電所_(Itami_Hendensho)/RConn3 -- L_110682955/LConn3
  T_185029969_500000;220000_/RConn1 -- L_185029969/LConn1
  T_185029969_500000;220000_/RConn2 -- L_185029969/LConn2
  T_185029969_500000;220000_/RConn3 -- L_185029969/LConn3
  T_170605907_500000_北摂変電所/RConn1 -- L_170605907/LConn1
  T_170605907_500000_北摂変電所/RConn2 -- L_170605907/LConn2
  T_170605907_500000_北摂変電所/RConn3 -- L_170605907/LConn3
  T_316459359_275000_/RConn1 -- L_316459359/LConn1
  T_316459359_275000_/RConn2 -- L_316459359/LConn2
  T_316459359_275000_/RConn3 -- L_316459359/LConn3
  T_144077272__/RConn1 -- L_144077272/LConn1
  T_144077272__/RConn2 -- L_144077272/LConn2
  T_144077272__/RConn3 -- L_144077272/LConn3
  T_152991099__中東京変電所/RConn1 -- L_152991099/LConn1
  T_152991099__中東京変電所/RConn2 -- L_152991099/LConn2
  T_152991099__中東京変電所/RConn3 -- L_152991099/LConn3
  T_190984572_275000_/RConn1 -- L_190984572/LConn1
  T_190984572_275000_/RConn2 -- L_190984572/LConn2
  T_190984572_275000_/RConn3 -- L_190984572/LConn3
  T_209726348_500000_信濃変電所/RConn1 -- L_209726348/LConn1
  T_209726348_500000_信濃変電所/RConn2 -- L_209726348/LConn2
  T_209726348_500000_信濃変電所/RConn3 -- L_209726348/LConn3
  T_209429410_500000_南信変電所/RConn1 -- L_209429410/LConn1
  T_209429410_500000_南信変電所/RConn2 -- L_209429410/LConn2
  T_209429410_500000_南信変電所/RConn3 -- L_209429410/LConn3
  T_315662839_500000_新信濃変電所/RConn1 -- L_315662839/LConn1
  T_315662839_500000_新信濃変電所/RConn2 -- L_315662839/LConn2
  T_315662839_500000_新信濃変電所/RConn3 -- L_315662839/LConn3
  T_217885658_500000;0_由良開閉所/RConn1 -- L_217885658/LConn1
  T_217885658_500000;0_由良開閉所/RConn2 -- L_217885658/LConn2
  T_217885658_500000;0_由良開閉所/RConn3 -- L_217885658/LConn3
  T_318302348_275000_東上越変電所/RConn1 -- L_318302348/LConn1
  T_318302348_275000_東上越変電所/RConn2 -- L_318302348/LConn2
  T_318302348_275000_東上越変電所/RConn3 -- L_318302348/LConn3
  T_153760214__多摩変電所/RConn1 -- L_153760214/LConn1
  T_153760214__多摩変電所/RConn2 -- L_153760214/LConn2
  T_153760214__多摩変電所/RConn3 -- L_153760214/LConn3
  T_315662816__/RConn1 -- L_315662816/LConn1
  T_315662816__/RConn2 -- L_315662816/LConn2
  T_315662816__/RConn3 -- L_315662816/LConn3
